simulink model "Library"  (R2020b)
settings: Solver=VariableStepAuto  StartTime=0.0  StopTime=2  RelTol=1e-3
settings Model: Creator=Stefano  LastModifiedBy=stefanopanzieri
settings SFSimCC: CustomCodeUndefinedFunction=UseInterfaceOnly

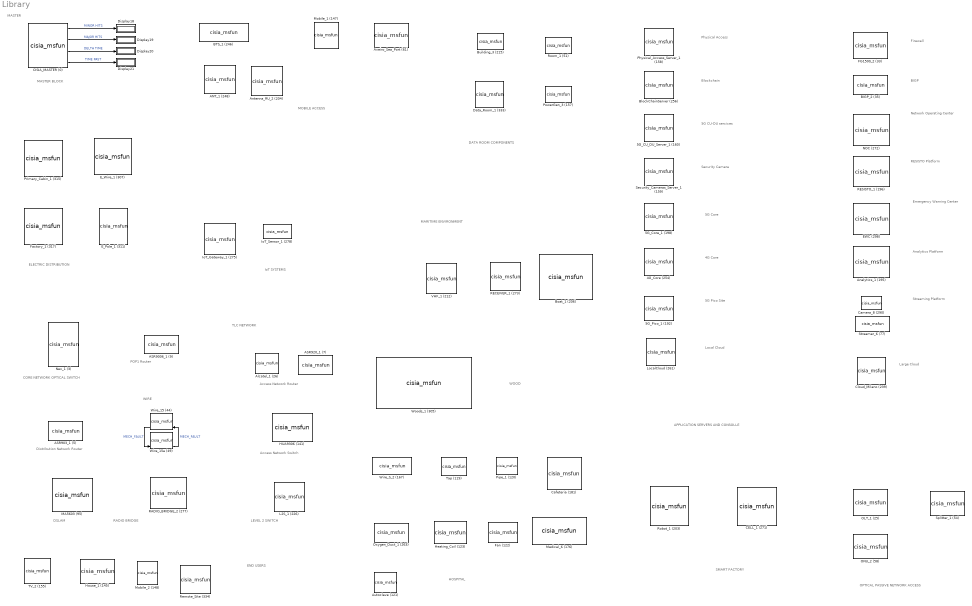
== system Library ==
  note: MASTER BLOCK
  note: MASTER
  note: ELECTRIC DISTRIBUTION
  note: TLC NETWORK
  note: MOBILE ACCESS
  note: MARITIME ENVIRONMENT
  note: DATA ROOM COMPONENTS
  note: APPLICATION SERVERS AND CONSOLLE
  note: IoT SYSTEMS
  note: SMART FACTORY
  note: HOSPITAL
  note: END USERS
  note: Access Network Router
  note: Access Network Switch
  note: Distribution Network Router
  note: DSLAM
  note: RADIO BRIDGE
  note: WIRE
  note: CORE NETWORK OPTICAL SWITCH
  note: POP1 Router
  note: LEVEL 2 SWITCH
  note: WOOD
  note: OPTICAL PASSIVE NETWORK ACCESS
  note: Physical Access
  note: Blockchain
  note: 5G CU-DU sercices
  note: Security Camera
  note: 5G Pico Site
  note: Large Cloud
  note: Local Cloud
  note: Firewall
  note: BIGP
  note: Network Operating Center
  note: RESISTO Platform
  note: Emergency Warning Center
  note: Analytics Platform
  note: Streaming Platform
  note: 4G Core
  note: 5G Core
  4G_Core (254) : M-S-Function  FunctionName=cisia_msfun  Parameters=Parameter1, Parameter2, Parameter3, resources, Parameter10, codeupdate, step_received, step_computed, dynamic_computed, step_sended, id_entity, id_project, id_type, name_type, color  mask(S-function:msfcn_unit_delay){Parameter1='4G_Core', Parameter2=1, Parameter3='ORO', resources=, Parameter10=off, codeupdate=off, step_received=|, step_computed=, dynamic_computed=, step_sended=|, id_entity=254, id_project=6, id_type=40, name_type=App_Server, color=#00AAFF}
      mask step_received=|
      | Connection=max(Connection_init,TLC_CONN);
      | TLC_services=max(TLC_services_init,TLC_SERVICE);
      | TLC_services=mod(TLC_services,10);
      | TLC_revoke=floor(TLC_SERVICE/10);
      |
      | Mechanical_Fault=max([Mechanical_Fault Mechanical_Fault_init]);
      |
      | %if strcmp(name_entity,"BlockChainServer") && (cisia.major_time>=2)
      |  % Dos_attack=1;
      |  %TLC_revoke(9)=1;
      |  %TLC_services(9)=0;
      | %end
      |
      |
      | Cyber_Fault=max(CYBER_FAULT, transpose([Dos_attack   MITM_attack Virus_Attack Port_Scan_Attack  BGP_hijacking BotNet_Attack Data_Corruption SW_Change Config_Change Port_Saturation]));
      |
      | Service_Fault=max(abs(Consumed_Services.*TLC_services-Consumed_Services));
      | Redundancy_Fault=max(abs(Consumed_Services.*TLC_CONN-Consumed_Services));
      |
      | Conn_Fault=max([Dos_attack  Mechanical_Fault  1-POWER 1-ROOM_QoS] );
      |
      |
      | Operative_Level=(1-Conn_Fault)*(1-0.5*max(Cyber_Fault))*(1-Service_Fault)*max(max(TLC_CONN),0.5);
      mask step_sended=|
      | TLC_CONN=Connection*(1-Conn_Fault);
      | TLC_SERVICE=TLC_services*(1-Conn_Fault)*(1-Service_Fault)*(1-syslog_adm_login)+10*TLC_revoke;
      | CYBER_FAULT=Cyber_Fault*(1-Conn_Fault);
      mask prompts: Parameter1 "entity name"; Parameter2 "sampling time"; Parameter3 "project"; resources "input resources and state variables"; Parameter10 "Bring state variables to output"; codeupdate "update code from mask"
      mask help: This is a level-2 MATLAB file S-function which demonstrates CISIA entity
      mask DialogControl Container1 Prompt: All parameters
      mask Display: image('Icons/App_Server.png')
  5G_CU_DU_Server_1 (160) : M-S-Function  FunctionName=cisia_msfun  Parameters=Parameter1, Parameter2, Parameter3, resources, Parameter10, codeupdate, step_received, step_computed, dynamic_computed, step_sended, id_entity, id_project, id_type, name_type, color  mask(S-function:msfcn_unit_delay){Parameter1='5G_CU_DU_Server_1', Parameter2=1, Parameter3='ORO', resources=, Parameter10=off, codeupdate=off, step_received=|, step_computed=, dynamic_computed=, step_sended=|, id_entity=160, id_project=6, id_type=40, name_type=App_Server, color=#00AAFF}
      mask step_received=|
      | Connection=max(Connection_init,TLC_CONN);
      | TLC_services=max(TLC_services_init,TLC_SERVICE);
      | TLC_services=mod(TLC_services,10);
      | TLC_revoke=floor(TLC_SERVICE/10);
      |
      | Mechanical_Fault=max([Mechanical_Fault Mechanical_Fault_init]);
      |
      | %if strcmp(name_entity,"BlockChainServer") && (cisia.major_time>=2)
      |  % Dos_attack=1;
      |  %TLC_revoke(9)=1;
      |  %TLC_services(9)=0;
      | %end
      |
      |
      | Cyber_Fault=max(CYBER_FAULT, transpose([Dos_attack   MITM_attack Virus_Attack Port_Scan_Attack  BGP_hijacking BotNet_Attack Data_Corruption SW_Change Config_Change Port_Saturation]));
      |
      | Service_Fault=max(abs(Consumed_Services.*TLC_services-Consumed_Services));
      | Redundancy_Fault=max(abs(Consumed_Services.*TLC_CONN-Consumed_Services));
      |
      | Conn_Fault=max([Dos_attack  Mechanical_Fault  1-POWER 1-ROOM_QoS] );
      |
      |
      | Operative_Level=(1-Conn_Fault)*(1-0.5*max(Cyber_Fault))*(1-Service_Fault)*max(max(TLC_CONN),0.5);
      mask step_sended=|
      | TLC_CONN=Connection*(1-Conn_Fault);
      | TLC_SERVICE=TLC_services*(1-Conn_Fault)*(1-Service_Fault)*(1-syslog_adm_login)+10*TLC_revoke;
      | CYBER_FAULT=Cyber_Fault*(1-Conn_Fault);
      mask prompts: Parameter1 "entity name"; Parameter2 "sampling time"; Parameter3 "project"; resources "input resources and state variables"; Parameter10 "Bring state variables to output"; codeupdate "update code from mask"
      mask help: This is a level-2 MATLAB file S-function which demonstrates CISIA entity
      mask DialogControl Container1 Prompt: All parameters
      mask Display: image('Icons/App_Server.png')
  5G_Core_1 (198) : M-S-Function  FunctionName=cisia_msfun  Parameters=Parameter1, Parameter2, Parameter3, resources, Parameter10, codeupdate, step_received, step_computed, dynamic_computed, step_sended, id_entity, id_project, id_type, name_type, color  mask(S-function:msfcn_unit_delay){Parameter1='5G_Core_1', Parameter2=1, Parameter3='ORO', resources=, Parameter10=off, codeupdate=off, step_received=|, step_computed=, dynamic_computed=, step_sended=|, id_entity=198, id_project=6, id_type=38, name_type=5G_Core, color=#E7A6FF}
      mask step_received=|
      | Connection=max(Connection_init,TLC_CONN);
      | TLC_services=max(TLC_services_init,TLC_SERVICE);
      | TLC_services=mod(TLC_services,10);
      | TLC_revoke=floor(TLC_SERVICE/10);
      | Mechanical_Fault=max([Mechanical_Fault Mechanical_Fault_init]);
      |
      | Cyber_Fault=max(CYBER_FAULT, transpose([Dos_attack   MITM_attack Virus_Attack Port_Scan_Attack  BGP_hijacking BotNet_Attack Data_Corruption SW_Change Config_Change Port_Saturation]));
      |
      |
      |
      | %if (cisia.major_time)>=2
      |    %Dos_attack=1;
      |    %TLC_services(5)=0;
      |   %TLC_revoke(5)=1;
      | %end
      |
      |
      | Conn_Fault=max([Dos_attack  Mechanical_Fault  1-POWER 1-ROOM_QoS] );
      |
      | Service_Fault=max(abs(Consumed_Services.*TLC_services-Consumed_Services));
      | Redundancy_Fault=max(abs(Consumed_Services.*TLC_CONN-Consumed_Services));
      |
      | Operative_Level=(1-Conn_Fault)*(1-0.5*max(Cyber_Fault))*(1-Service_Fault);
      mask step_sended=|
      | TLC_CONN=Connection*(1-Conn_Fault);
      | TLC_SERVICE=TLC_services*(1-Conn_Fault)*(1-Service_Fault)*(1 -syslog_adm_login)+10*TLC_revoke;
      | %TLC_SERVICE=TLC_services
      | CYBER_FAULT=Cyber_Fault*(1-Conn_Fault);
      mask prompts: Parameter1 "entity name"; Parameter2 "sampling time"; Parameter3 "project"; resources "input resources and state variables"; Parameter10 "Bring state variables to output"; codeupdate "update code from mask"
      mask help: This is a level-2 MATLAB file S-function which demonstrates CISIA entity
      mask DialogControl Container1 Prompt: All parameters
      mask Display: image('Icons/5G_Core.png')
  5G_Pico_1 (192) : M-S-Function  FunctionName=cisia_msfun  Parameters=Parameter1, Parameter2, Parameter3, resources, Parameter10, codeupdate, step_received, step_computed, dynamic_computed, step_sended, id_entity, id_project, id_type, name_type, color  mask(S-function:msfcn_unit_delay){Parameter1='5G_Pico_1', Parameter2=1, Parameter3='ORO', resources=, Parameter10=off, codeupdate=off, step_received=|, step_computed=, dynamic_computed=, step_sended=|, id_entity=192, id_project=6, id_type=42, name_type=5G_CU_DU, color=#FF00FF}
      mask step_received=|
      | Connection=max(Connection_init,TLC_CONN);
      | TLC_services=max(TLC_services_init,TLC_SERVICE);
      | TLC_services=mod(TLC_services,10);
      | TLC_revoke=floor(TLC_SERVICE/10);
      |
      | Cyber_Fault=max(CYBER_FAULT, transpose([Dos_attack   MITM_attack Virus_Attack Port_Scan_Attack  BGP_hijacking BotNet_Attack Data_Corruption SW_Change Config_Change Port_Saturation]));
      |
      | Conn_Fault=max([Dos_attack  Mechanical_Fault  1-POWER 1-ROOM_QoS] );
      |
      | Service_Fault=max(abs(Consumed_Services.*TLC_services-Consumed_Services));
      | Redundancy_Fault=max(abs(Consumed_Services.*TLC_CONN-Consumed_Services));
      |
      | Operative_Level=(1-Conn_Fault)*(1-0.5*max(Cyber_Fault))*(1-Service_Fault)*max(max(TLC_CONN),0.5);
      mask step_sended=|
      | TLC_CONN=Connection*(1-Conn_Fault);
      | TLC_SERVICE=TLC_services*(1-Conn_Fault)*(1-Service_Fault)+TLC_revoke*10;
      | CYBER_FAULT=Cyber_Fault*(1-Conn_Fault);
      mask prompts: Parameter1 "entity name"; Parameter2 "sampling time"; Parameter3 "project"; resources "input resources and state variables"; Parameter10 "Bring state variables to output"; codeupdate "update code from mask"
      mask help: This is a level-2 MATLAB file S-function which demonstrates CISIA entity
      mask DialogControl Container1 Prompt: All parameters
      mask Display: disp('5G_CU_DU')
  ANT_1 (248) : M-S-Function  FunctionName=cisia_msfun  Parameters=Parameter1, Parameter2, Parameter3, resources, Parameter10, codeupdate, step_received, step_computed, dynamic_computed, step_sended, id_entity, id_project, id_type, name_type, color  mask(S-function:msfcn_unit_delay){Parameter1='ANT_1', Parameter2=1, Parameter3='ORO', resources=, Parameter10=off, codeupdate=off, step_received=|, step_computed=, dynamic_computed=, step_sended=|, id_entity=248, id_project=6, id_type=55, name_type=BTS_ANTENNA, color=#FFFFFF}
      mask step_received=|
      | Connection=max(Connection_init,BTS_CONN);
      | TLC_services=max(TLC_services_init,TLC_SERVICE);
      | TLC_services=mod(TLC_services,10);
      | TLC_revoke=floor(TLC_SERVICE/10);
      |
      | Cyber_Fault=max(CYBER_FAULT, transpose([Dos_attack   MITM_attack Virus_Attack Port_Scan_Attack  BGP_hijacking BotNet_Attack Data_Corruption SW_Change Config_Change Port_Saturation]));
      |
      | Conn_Fault=max([Dos_attack  Mechanical_Fault  1-POWER] );
      |
      | Service_Fault=max(abs(Consumed_Services.*TLC_services-Consumed_Services));
      | Redundancy_Fault=max(abs(Consumed_Services.*BTS_CONN-Consumed_Services));
      |
      | Operative_Level=(1-Conn_Fault)*(1-0.5*max(Cyber_Fault))*(1-Service_Fault);
      |
      | %Operative_Level=(1-Conn_Fault)*((2*(1-Service_Fault)+(1-Redundancy_Fault))/3);
      | %Operative_Level=(1-Conn_Fault)*max(max(BTS_CONN),0.5)*((2*(1-Service_Fault)+(1-Redundancy_Fault))/3);
      |
      | % Il servizio utilizzato
      | %My_Service=max([(1-Service_Fault) (1-Redundancy_Fault)/2]);
      mask step_sended=|
      | R_CONN=Connection*(1-Conn_Fault);
      | TLC_SERVICE=TLC_services*(1-Conn_Fault)*(1-Service_Fault)+10*TLC_revoke;
      | CYBER_FAULT=Cyber_Fault*(1-Conn_Fault);
      mask prompts: Parameter1 "entity name"; Parameter2 "sampling time"; Parameter3 "project"; resources "input resources and state variables"; Parameter10 "Bring state variables to output"; codeupdate "update code from mask"
      mask help: This is a level-2 MATLAB file S-function which demonstrates CISIA entity
      mask DialogControl Container1 Prompt: All parameters
      mask Display: image('Icons/BTS_ANTENNA.png')
  ASR9006_1 (9) : M-S-Function  FunctionName=cisia_msfun  Parameters=Parameter1, Parameter2, Parameter3, resources, Parameter10, codeupdate, step_received, step_computed, dynamic_computed, step_sended, id_entity, id_project, id_type, name_type, color  mask(S-function:msfcn_unit_delay){Parameter1='ASR9006_1', Parameter2=1, Parameter3='ORO', resources=, Parameter10=off, codeupdate=off, step_received=|, step_computed=, dynamic_computed=, step_sended=|, id_entity=9, id_project=6, id_type=3, name_type=CISCO_router, color=#4DBEEE}
      mask step_received=|
      | Connection=max(Connection_init,TLC_CONN);
      | TLC_services=max(TLC_services_init,TLC_SERVICE);
      | TLC_services=mod(TLC_services,10);
      | TLC_revoke=floor(TLC_SERVICE/10);
      |
      | Cyber_Fault=max(CYBER_FAULT, transpose([Dos_attack   MITM_attack Virus_Attack Port_Scan_Attack  BGP_hijacking BotNet_Attack Data_Corruption SW_Change Config_Change Port_Saturation]));
      |
      |
      | Conn_Fault=max([Dos_attack BGP_hijacking Route_Poisoning Interface_Down Mechanical_Fault  1-POWER 1-ROOM_QoS Earthquake_Fault] );
      |
      | Room_Fault=1-ROOM_QoS;
      |
      | Operative_Level=(1-Room_Fault)*(1-Conn_Fault)*max(max(TLC_services),0.5)*(1-0.5*max(Cyber_Fault));
      mask step_sended=|
      | TLC_CONN=Connection*(1-Conn_Fault);
      | TLC_SERVICE=TLC_services*(1-Room_Fault)*(1-Conn_Fault)*(1-syslog_adm_login)+10*TLC_revoke;
      |
      |
      | Cyber_Transmitted=min(Cyber_Fault, transpose([0 0 1 0 1 1 0 0 0 1]));
      |
      | CYBER_FAULT=Cyber_Transmitted*(1-Conn_Fault);
      |
      | ROUTING_QoS=Operative_Level;
      mask prompts: Parameter1 "entity name"; Parameter2 "sampling time"; Parameter3 "project"; resources "input resources and state variables"; Parameter10 "Bring state variables to output"; codeupdate "update code from mask"
      mask help: This is a level-2 MATLAB file S-function which demonstrates CISIA entity
      mask DialogControl Container1 Prompt: All parameters
      mask Display: image('Icons/CISCO_router.png')
  ASR903_1 (5) : M-S-Function  FunctionName=cisia_msfun  Parameters=Parameter1, Parameter2, Parameter3, resources, Parameter10, codeupdate, step_received, step_computed, dynamic_computed, step_sended, id_entity, id_project, id_type, name_type, color  mask(S-function:msfcn_unit_delay){Parameter1='ASR903_1', Parameter2=1, Parameter3='ORO', resources=, Parameter10=off, codeupdate=off, step_received=|, step_computed=, dynamic_computed=, step_sended=|, id_entity=5, id_project=6, id_type=3, name_type=CISCO_router, color=#4DBEEE}
      mask step_received=|
      | Connection=max(Connection_init,TLC_CONN);
      | TLC_services=max(TLC_services_init,TLC_SERVICE);
      | TLC_services=mod(TLC_services,10);
      | TLC_revoke=floor(TLC_SERVICE/10);
      |
      | Cyber_Fault=max(CYBER_FAULT, transpose([Dos_attack   MITM_attack Virus_Attack Port_Scan_Attack  BGP_hijacking BotNet_Attack Data_Corruption SW_Change Config_Change Port_Saturation]));
      |
      |
      | Conn_Fault=max([Dos_attack BGP_hijacking Route_Poisoning Interface_Down Mechanical_Fault  1-POWER 1-ROOM_QoS Earthquake_Fault] );
      |
      | Room_Fault=1-ROOM_QoS;
      |
      | Operative_Level=(1-Room_Fault)*(1-Conn_Fault)*max(max(TLC_services),0.5)*(1-0.5*max(Cyber_Fault));
      mask step_sended=|
      | TLC_CONN=Connection*(1-Conn_Fault);
      | TLC_SERVICE=TLC_services*(1-Room_Fault)*(1-Conn_Fault)*(1-syslog_adm_login)+10*TLC_revoke;
      |
      |
      | Cyber_Transmitted=min(Cyber_Fault, transpose([0 0 1 0 1 1 0 0 0 1]));
      |
      | CYBER_FAULT=Cyber_Transmitted*(1-Conn_Fault);
      |
      | ROUTING_QoS=Operative_Level;
      mask prompts: Parameter1 "entity name"; Parameter2 "sampling time"; Parameter3 "project"; resources "input resources and state variables"; Parameter10 "Bring state variables to output"; codeupdate "update code from mask"
      mask help: This is a level-2 MATLAB file S-function which demonstrates CISIA entity
      mask DialogControl Container1 Prompt: All parameters
      mask Display: image('Icons/CISCO_router.png')
  ASR920_1 (7) : M-S-Function  FunctionName=cisia_msfun  Parameters=Parameter1, Parameter2, Parameter3, resources, Parameter10, codeupdate, step_received, step_computed, dynamic_computed, step_sended, id_entity, id_project, id_type, name_type, color  mask(S-function:msfcn_unit_delay){Parameter1='ASR920_1', Parameter2=1, Parameter3='ORO', resources=, Parameter10=off, codeupdate=off, step_received=|, step_computed=, dynamic_computed=, step_sended=|, id_entity=7, id_project=6, id_type=3, name_type=CISCO_router, color=#4DBEEE}
      mask step_received=|
      | Connection=max(Connection_init,TLC_CONN);
      | TLC_services=max(TLC_services_init,TLC_SERVICE);
      | TLC_services=mod(TLC_services,10);
      | TLC_revoke=floor(TLC_SERVICE/10);
      |
      | Cyber_Fault=max(CYBER_FAULT, transpose([Dos_attack   MITM_attack Virus_Attack Port_Scan_Attack  BGP_hijacking BotNet_Attack Data_Corruption SW_Change Config_Change Port_Saturation]));
      |
      |
      | Conn_Fault=max([Dos_attack BGP_hijacking Route_Poisoning Interface_Down Mechanical_Fault  1-POWER 1-ROOM_QoS Earthquake_Fault] );
      |
      | Room_Fault=1-ROOM_QoS;
      |
      | Operative_Level=(1-Room_Fault)*(1-Conn_Fault)*max(max(TLC_services),0.5)*(1-0.5*max(Cyber_Fault));
      mask step_sended=|
      | TLC_CONN=Connection*(1-Conn_Fault);
      | TLC_SERVICE=TLC_services*(1-Room_Fault)*(1-Conn_Fault)*(1-syslog_adm_login)+10*TLC_revoke;
      |
      |
      | Cyber_Transmitted=min(Cyber_Fault, transpose([0 0 1 0 1 1 0 0 0 1]));
      |
      | CYBER_FAULT=Cyber_Transmitted*(1-Conn_Fault);
      |
      | ROUTING_QoS=Operative_Level;
      mask prompts: Parameter1 "entity name"; Parameter2 "sampling time"; Parameter3 "project"; resources "input resources and state variables"; Parameter10 "Bring state variables to output"; codeupdate "update code from mask"
      mask help: This is a level-2 MATLAB file S-function which demonstrates CISIA entity
      mask DialogControl Container1 Prompt: All parameters
      mask Display: image('Icons/CISCO_router.png')
  Alcatel_1 (26) : M-S-Function  FunctionName=cisia_msfun  Parameters=Parameter1, Parameter2, Parameter3, resources, Parameter10, codeupdate, step_received, step_computed, dynamic_computed, step_sended, id_entity, id_project, id_type, name_type, color  mask(S-function:msfcn_unit_delay){Parameter1='Alcatel_1', Parameter2=1, Parameter3='ORO', resources=, Parameter10=off, codeupdate=off, step_received=|, step_computed=, dynamic_computed=, step_sended=|, id_entity=26, id_project=6, id_type=5, name_type=Alcatel7750, color=#ACBD7E}
      mask step_received=|
      | Connection=max(Connection_init,TLC_CONN);
      | TLC_services=max(TLC_services_init,TLC_SERVICE);
      | TLC_services=mod(TLC_services,10);
      | TLC_revoke=floor(TLC_SERVICE/10);
      |
      | Cyber_Fault=max(CYBER_FAULT, transpose([Dos_attack   MITM_attack Virus_Attack Port_Scan_Attack  BGP_hijacking BotNet_Attack Data_Corruption SW_Change Config_Change Port_Saturation]));
      |
      | Conn_Fault=max([Dos_attack  Mechanical_Fault  1-POWER 1-ROOM_QoS] );
      |
      |
      | Operative_Level=(1-Conn_Fault)*(1-0.5*max(Cyber_Fault))*max(max(TLC_services),0.5);
      mask step_sended=|
      | TLC_CONN=Connection*(1-Conn_Fault);
      | TLC_SERVICE=TLC_services*(1-Conn_Fault)+TLC_revoke*10;
      | CYBER_FAULT=Cyber_Fault*(1-Conn_Fault);
      |
      | ROUTING_QoS=Operative_Level;
      mask prompts: Parameter1 "entity name"; Parameter2 "sampling time"; Parameter3 "project"; resources "input resources and state variables"; Parameter10 "Bring state variables to output"; codeupdate "update code from mask"
      mask help: This is a level-2 MATLAB file S-function which demonstrates CISIA entity
      mask DialogControl Container1 Prompt: All parameters
      mask Display: image('Icons/Alcatel7750.png')
  Analytics_1 (195) : M-S-Function  FunctionName=cisia_msfun  Parameters=Parameter1, Parameter2, Parameter3, resources, Parameter10, codeupdate, step_received, step_computed, dynamic_computed, step_sended, id_entity, id_project, id_type, name_type, color  mask(S-function:msfcn_unit_delay){Parameter1='Analytics_1', Parameter2=1, Parameter3='ORO', resources=, Parameter10=off, codeupdate=off, step_received=|, step_computed=, dynamic_computed=, step_sended=WORKSTATION_QoS=Operative_Level;, id_entity=195, id_project=6, id_type=43, name_type=Workstation, color=#FFFFFF}
      mask step_received=|
      | Connection=max(Connection_init,TLC_CONN);
      |
      | Cyber_Fault=max(CYBER_FAULT, transpose([Dos_attack   MITM_attack Virus_Attack Port_Scan_Attack  BGP_hijacking BotNet_Attack Data_Corruption SW_Change Config_Change Port_Saturation]));
      |
      | % Vale 1 in presenza di fault
      | Conn_Fault=max([Dos_attack  Mechanical_Fault  1-POWER] );
      |
      |
      |
      | Operative_Level=(1-Conn_Fault)*max(max(TLC_CONN),0.5);
      mask prompts: Parameter1 "entity name"; Parameter2 "sampling time"; Parameter3 "project"; resources "input resources and state variables"; Parameter10 "Bring state variables to output"; codeupdate "update code from mask"
      mask help: This is a level-2 MATLAB file S-function which demonstrates CISIA entity
      mask DialogControl Container1 Prompt: All parameters
      mask Display: image('Icons/Analytics_1.png')
  Antenna_RU_2 (204) : M-S-Function  FunctionName=cisia_msfun  Parameters=Parameter1, Parameter2, Parameter3, resources, Parameter10, codeupdate, step_received, step_computed, dynamic_computed, step_sended, id_entity, id_project, id_type, name_type, color  mask(S-function:msfcn_unit_delay){Parameter1='Antenna_RU_2', Parameter2=1, Parameter3='ORO', resources=, Parameter10=off, codeupdate=off, step_received=|, step_computed=, dynamic_computed=, step_sended=|, id_entity=204, id_project=6, id_type=41, name_type=RU_ANTENNA, color=#FFFFFF}
      mask step_received=|
      | Connection=max(Connection_init,TLC_CONN);
      | TLC_services=max(TLC_services_init,TLC_SERVICE);
      | TLC_services=mod(TLC_services,10);
      | TLC_revoke=floor(TLC_SERVICE/10);
      |
      | Cyber_Fault=max(CYBER_FAULT, transpose([Dos_attack   MITM_attack Virus_Attack Port_Scan_Attack  BGP_hijacking BotNet_Attack Data_Corruption SW_Change Config_Change Port_Saturation]));
      |
      | % Vale 1 in presenza di fault
      | Conn_Fault=max([Dos_attack  Mechanical_Fault  1-POWER] );
      |
      | Service_Fault=max(abs(Consumed_Services.*TLC_services-Consumed_Services));
      | Redundancy_Fault=max(abs(Consumed_Services.*TLC_CONN-Consumed_Services));
      |
      |
      | Operative_Level=(1-Conn_Fault)*max(max(TLC_services),0.5)*(1-Service_Fault)*(1-0.5*max(Cyber_Fault))*max(max(TLC_CONN),0.5);
      |
      | % Il servizio utilizzato
      | %My_Service=max([(1-Service_Fault) (1-Redundancy_Fault)/2]);
      mask step_sended=|
      | R_CONN=Connection*(1-Conn_Fault);
      | TLC_SERVICE=TLC_services*(1-Conn_Fault)+10*TLC_revoke;
      |
      | Cyber_Transmitted=min(Cyber_Fault, transpose([0 0 1 0 1 1 0 0 0 1]));
      | CYBER_FAULT=Cyber_Transmitted*(1-Conn_Fault);
      mask prompts: Parameter1 "entity name"; Parameter2 "sampling time"; Parameter3 "project"; resources "input resources and state variables"; Parameter10 "Bring state variables to output"; codeupdate "update code from mask"
      mask help: This is a level-2 MATLAB file S-function which demonstrates CISIA entity
      mask DialogControl Container1 Prompt: All parameters
      mask Display: image('Icons/RU_ANTENNA.png')
  Autoclave (121) : M-S-Function  FunctionName=cisia_msfun  Parameters=Parameter1, Parameter2, Parameter3, resources, Parameter10, codeupdate, step_received, step_computed, dynamic_computed, step_sended, id_entity, id_project, id_type, name_type, color  mask(S-function:msfcn_unit_delay){Parameter1='Autoclave', Parameter2=1, Parameter3='ORO', resources=, Parameter10=off, codeupdate=off, step_received=|, step_computed=, dynamic_computed=, step_sended=WATER=Operative_Level;, id_entity=121, id_project=6, id_type=33, name_type=Autoclave, color=#FFFFFF}
      mask step_received=|
      | Water_Fault=1-WATER;
      | Power_Fault=1-POWER;
      |
      | Operative_Level=min([ 1-Mechanical_Fault 1-Power_Fault 1-Water_Fault]);
      mask prompts: Parameter1 "entity name"; Parameter2 "sampling time"; Parameter3 "project"; resources "input resources and state variables"; Parameter10 "Bring state variables to output"; codeupdate "update code from mask"
      mask help: This is a level-2 MATLAB file S-function which demonstrates CISIA entity
      mask DialogControl Container1 Prompt: All parameters
      mask Display: disp('Autoclave')
  Aveiro_Sea_Port (61) : M-S-Function  FunctionName=cisia_msfun  Parameters=Parameter1, Parameter2, Parameter3, resources, Parameter10, codeupdate, step_received, step_computed, dynamic_computed, step_sended, id_entity, id_project, id_type, name_type, color  mask(S-function:msfcn_unit_delay){Parameter1='Aveiro_Sea_Port', Parameter2=1, Parameter3='ORO', resources=, Parameter10=off, codeupdate=off, step_received=|, step_computed=, dynamic_computed=, step_sended=|, id_entity=61, id_project=6, id_type=14, name_type=Cell_Area, color=#0FFFFF}
      mask step_received=|
      | Connection=max(Connection_init,R_CONN);
      | TLC_services=max(TLC_services_init,TLC_SERVICE);
      | TLC_services=mod(TLC_services,10);
      | TLC_revoke=floor(TLC_SERVICE/10);
      |
      | Cyber_Fault=max(CYBER_FAULT, transpose([Dos_attack   MITM_attack Virus_Attack Port_Scan_Attack  BGP_hijacking BotNet_Attack Data_Corruption SW_Change Config_Change Port_Saturation]));
      |
      | % Vale 1 in presenza di fault
      | Conn_Fault=max([Dos_attack  Mechanical_Fault] );
      |
      | Service_Fault=max(abs(Consumed_Services.*TLC_services-Consumed_Services));
      | Redundancy_Fault=max(abs(Consumed_Services.*R_CONN-Consumed_Services));
      |
      |
      | Operative_Level=(1-Conn_Fault)*max(max(R_CONN),0.5)*((2*(1-Service_Fault)+(1-Redundancy_Fault))/3);
      |
      | % Il servizio utilizzato
      | My_Service=max([(1-Service_Fault) (1-Redundancy_Fault)/2]);
      mask step_sended=|
      | R_CONN=Connection*(1-Conn_Fault);
      | TLC_SERVICE=TLC_services*(1-Conn_Fault)+10*TLC_revoke;
      | CYBER_FAULT=Cyber_Fault*(1-Conn_Fault);
      |
      | CELL_QoS=My_Service;
      mask prompts: Parameter1 "entity name"; Parameter2 "sampling time"; Parameter3 "project"; resources "input resources and state variables"; Parameter10 "Bring state variables to output"; codeupdate "update code from mask"
      mask help: This is a level-2 MATLAB file S-function which demonstrates CISIA entity
      mask DialogControl Container1 Prompt: All parameters
      mask Display: disp('Cell_Area')
  BIGP_2 (35) : M-S-Function  FunctionName=cisia_msfun  Parameters=Parameter1, Parameter2, Parameter3, resources, Parameter10, codeupdate, step_received, step_computed, dynamic_computed, step_sended, id_entity, id_project, id_type, name_type, color  mask(S-function:msfcn_unit_delay){Parameter1='BIGP_2', Parameter2=1, Parameter3='ORO', resources=, Parameter10=off, codeupdate=off, step_received=|, step_computed=, dynamic_computed=, step_sended=|, id_entity=35, id_project=6, id_type=7, name_type=F5BIGP, color=#0072BD}
      mask step_received=|
      | Connection=max(Connection_init,TLC_CONN);
      | TLC_services=max(TLC_services_init,TLC_SERVICE);
      | TLC_services=mod(TLC_services,10);
      | TLC_revoke=floor(TLC_SERVICE/10);
      |
      | Cyber_Fault=max(CYBER_FAULT, transpose([Dos_attack   MITM_attack Virus_Attack Port_Scan_Attack  BGP_hijacking BotNet_Attack Data_Corruption SW_Change Config_Change Port_Saturation]));
      |
      | Conn_Fault=max([Dos_attack  Mechanical_Fault  1-POWER 1-ROOM_QoS] );
      |
      | Service_Fault=max(abs(Consumed_Services.*TLC_services-Consumed_Services));
      | Redundancy_Fault=max(abs(Consumed_Services.*TLC_CONN-Consumed_Services));
      |
      | %Operative_Level=(1-Conn_Fault)*((2*(1-Service_Fault)+(1-Redundancy_Fault))/3);
      | Operative_Level=(1-Conn_Fault)*(1-0.5*max(Cyber_Fault))*(1-Service_Fault)*max(max(TLC_CONN),0.5);
      mask step_sended=|
      | TLC_CONN=Connection*(1-Conn_Fault);
      | TLC_SERVICE=TLC_services*(1-Conn_Fault)*(1-Service_Fault)+10*TLC_revoke;
      |
      | Cyber_Transmitted=min(Cyber_Fault, transpose([0 0 1 0 1 1 0 0 0 1]));
      |
      | CYBER_FAULT=Cyber_Transmitted*(1-Conn_Fault);
      mask prompts: Parameter1 "entity name"; Parameter2 "sampling time"; Parameter3 "project"; resources "input resources and state variables"; Parameter10 "Bring state variables to output"; codeupdate "update code from mask"
      mask help: This is a level-2 MATLAB file S-function which demonstrates CISIA entity
      mask DialogControl Container1 Prompt: All parameters
      mask Display: disp('F5BIGP')
  BTS_1 (246) : M-S-Function  FunctionName=cisia_msfun  Parameters=Parameter1, Parameter2, Parameter3, resources, Parameter10, codeupdate, step_received, step_computed, dynamic_computed, step_sended, id_entity, id_project, id_type, name_type, color  mask(S-function:msfcn_unit_delay){Parameter1='BTS_1', Parameter2=1, Parameter3='ORO', resources=, Parameter10=off, codeupdate=off, step_received=|, step_computed=, dynamic_computed=, step_sended=|, id_entity=246, id_project=6, id_type=54, name_type=BaseTransceiverStation, color=#FFFFFF}
      mask step_received=|
      | Connection=max(Connection_init,TLC_CONN);
      | TLC_services=max(TLC_services_init,TLC_SERVICE);
      | TLC_services=mod(TLC_services,10);
      | TLC_revoke=floor(TLC_SERVICE/10);
      |
      | Cyber_Fault=max(CYBER_FAULT, transpose([Dos_attack   MITM_attack Virus_Attack Port_Scan_Attack  BGP_hijacking BotNet_Attack Data_Corruption SW_Change Config_Change Port_Saturation]));
      |
      | Conn_Fault=max([Dos_attack  Mechanical_Fault ] );
      |
      | Operative_Level=(1-Conn_Fault)*max(max(TLC_services),0.5)*(1-0.5*max(Cyber_Fault));
      mask step_sended=|
      | BTS_CONN=Connection*(1-Conn_Fault);
      | TLC_SERVICE=TLC_services*(1-Conn_Fault)+10*TLC_revoke;
      | CYBER_FAULT=Cyber_Fault*(1-Conn_Fault);
      mask prompts: Parameter1 "entity name"; Parameter2 "sampling time"; Parameter3 "project"; resources "input resources and state variables"; Parameter10 "Bring state variables to output"; codeupdate "update code from mask"
      mask help: This is a level-2 MATLAB file S-function which demonstrates CISIA entity
      mask DialogControl Container1 Prompt: All parameters
      mask Display: disp('BaseTransceiverStation')
  BlockChainServer (256) : M-S-Function  FunctionName=cisia_msfun  Parameters=Parameter1, Parameter2, Parameter3, resources, Parameter10, codeupdate, step_received, step_computed, dynamic_computed, step_sended, id_entity, id_project, id_type, name_type, color  mask(S-function:msfcn_unit_delay){Parameter1='BlockChainServer', Parameter2=1, Parameter3='ORO', resources=, Parameter10=on, codeupdate=off, step_received=|, step_computed=, dynamic_computed=, step_sended=|, id_entity=256, id_project=6, id_type=40, name_type=App_Server, color=#00AAFF}
      mask step_received=|
      | Connection=max(Connection_init,TLC_CONN);
      | TLC_services=max(TLC_services_init,TLC_SERVICE);
      | TLC_services=mod(TLC_services,10);
      | TLC_revoke=floor(TLC_SERVICE/10);
      |
      | Mechanical_Fault=max([Mechanical_Fault Mechanical_Fault_init]);
      |
      | %if strcmp(name_entity,"BlockChainServer") && (cisia.major_time>=2)
      |  % Dos_attack=1;
      |  %TLC_revoke(9)=1;
      |  %TLC_services(9)=0;
      | %end
      |
      |
      | Cyber_Fault=max(CYBER_FAULT, transpose([Dos_attack   MITM_attack Virus_Attack Port_Scan_Attack  BGP_hijacking BotNet_Attack Data_Corruption SW_Change Config_Change Port_Saturation]));
      |
      | Service_Fault=max(abs(Consumed_Services.*TLC_services-Consumed_Services));
      | Redundancy_Fault=max(abs(Consumed_Services.*TLC_CONN-Consumed_Services));
      |
      | Conn_Fault=max([Dos_attack  Mechanical_Fault  1-POWER 1-ROOM_QoS] );
      |
      |
      | Operative_Level=(1-Conn_Fault)*(1-0.5*max(Cyber_Fault))*(1-Service_Fault)*max(max(TLC_CONN),0.5);
      mask step_sended=|
      | TLC_CONN=Connection*(1-Conn_Fault);
      | TLC_SERVICE=TLC_services*(1-Conn_Fault)*(1-Service_Fault)*(1-syslog_adm_login)+10*TLC_revoke;
      | CYBER_FAULT=Cyber_Fault*(1-Conn_Fault);
      mask prompts: Parameter1 "entity name"; Parameter2 "sampling time"; Parameter3 "project"; resources "input resources and state variables"; Parameter10 "Bring state variables to output"; codeupdate "update code from mask"
      mask help: This is a level-2 MATLAB file S-function which demonstrates CISIA entity
      mask DialogControl Container1 Prompt: All parameters
      mask Display: image('Icons/App_Server.png')
  Boat_1 (206) : M-S-Function  FunctionName=cisia_msfun  Parameters=Parameter1, Parameter2, Parameter3, resources, Parameter10, codeupdate, step_received, step_computed, dynamic_computed, step_sended, id_entity, id_project, id_type, name_type, color  mask(S-function:msfcn_unit_delay){Parameter1='Boat_1', Parameter2=1, Parameter3='ORO', resources=, Parameter10=off, codeupdate=off, step_received=|, step_computed=, dynamic_computed=, step_sended=|, id_entity=206, id_project=6, id_type=45, name_type=Boat, color=#FFFFFF}
      mask step_received=|
      | Conn_Fault=1-max(VDES_CONN,AIS_CONN);
      |
      |
      | Operative_Level=(1-Mechanical_Fault)*(1-Conn_Fault);
      mask step_sended=|
      | BOAT_QoS=Operative_Level;
      | AIS_CON=1-Conn_Fault;
      | VDES_CONN=1-Conn_Fault;
      mask prompts: Parameter1 "entity name"; Parameter2 "sampling time"; Parameter3 "project"; resources "input resources and state variables"; Parameter10 "Bring state variables to output"; codeupdate "update code from mask"
      mask help: This is a level-2 MATLAB file S-function which demonstrates CISIA entity
      mask DialogControl Container1 Prompt: All parameters
      mask Display: image('Icons/Boat.png')
  Building_3 (215) : M-S-Function  FunctionName=cisia_msfun  Parameters=Parameter1, Parameter2, Parameter3, resources, Parameter10, codeupdate, step_received, step_computed, dynamic_computed, step_sended, id_entity, id_project, id_type, name_type, color  mask(S-function:msfcn_unit_delay){Parameter1='Building_3', Parameter2=1, Parameter3='ORO', resources=, Parameter10=off, codeupdate=off, step_received=|, step_computed=, dynamic_computed=, step_sended=|, id_entity=215, id_project=6, id_type=10, name_type=Building, color=#AB7A07}
      mask step_received=|
      | Physical_Fault=max([Unauthorized_Access Perimeter_Security_Fault Security_Camera_Fault Earthquake_Fault]);
      |
      | Conn_Fault=max([Power_Fault 1-ROOM_QoS]);
      |
      | Operative_Level=min([ (1-Physical_Fault) (1-Conn_Fault) (1-Perimeter_Security_Fault) (1-Earthquake_Fault) ]);
      mask step_sended=|
      | BUILDING_QoS=Operative_Level;
      |
      | %Cyber_Fault=0.3*ones(size(Cyber_Fault));
      |
      | CYBER_FAULT=Perimeter_Security_Fault*Cyber_Fault;
      mask prompts: Parameter1 "entity name"; Parameter2 "sampling time"; Parameter3 "project"; resources "input resources and state variables"; Parameter10 "Bring state variables to output"; codeupdate "update code from mask"
      mask help: This is a level-2 MATLAB file S-function which demonstrates CISIA entity
      mask DialogControl Container1 Prompt: All parameters
      mask Display: image('Icons/Building.png')
  CELL_1 (271) : M-S-Function  FunctionName=cisia_msfun  Parameters=Parameter1, Parameter2, Parameter3, resources, Parameter10, codeupdate, step_received, step_computed, dynamic_computed, step_sended, id_entity, id_project, id_type, name_type, color  mask(S-function:msfcn_unit_delay){Parameter1='CELL_1', Parameter2=1, Parameter3='ORO', resources=, Parameter10=off, codeupdate=off, step_received=Operative_Level=ROBOT_QoS;, step_computed=, dynamic_computed=, step_sended=WORKING_CELL_QoS=Operative_Level;, id_entity=271, id_project=6, id_type=58, name_type=Working_Cell, color=#00FFAA}
      mask prompts: Parameter1 "entity name"; Parameter2 "sampling time"; Parameter3 "project"; resources "input resources and state variables"; Parameter10 "Bring state variables to output"; codeupdate "update code from mask"
      mask help: This is a level-2 MATLAB file S-function which demonstrates CISIA entity
      mask DialogControl Container1 Prompt: All parameters
      mask Display: image('Icons/Working_Cell.png')
  CISIA_MASTER (0) : M-S-Function  FunctionName=cisia_msfun  Parameters=Parameter1, Parameter2, Parameter3, resources, Parameter4, Parameter5, Parameter6, Parameter7, Parameter8, Parameter9  mask(S-function:msfcn_unit_delay){Parameter1='CISIA_MASTER', Parameter2=0.001, Parameter3='ORO', resources=off, Parameter4=on, Parameter5=off, Parameter6=off, Parameter7=off, Parameter8=1, Parameter9=off}
      mask prompts: Parameter1 "entity name"; Parameter2 "sampling time"; Parameter3 "project"; resources "Save status at each major hit"; Parameter4 "Show Operative Levels with colors"; Parameter5 "Load Entities from file"; Parameter6 "Load Start from Mask"; Parameter7 "Real Time"; Parameter8 "Real Time Hit (sec)"; Parameter9 "Skip saving"
      mask help: This is a level-2 MATLAB file S-function which demonstrates CISIA entity
      mask Display: disp('MASTER BLOCK')
  Cafeteria (181) : M-S-Function  FunctionName=cisia_msfun  Parameters=Parameter1, Parameter2, Parameter3, resources, Parameter10, codeupdate, step_received, step_computed, dynamic_computed, step_sended, id_entity, id_project, id_type, name_type, color  mask(S-function:msfcn_unit_delay){Parameter1='Cafeteria', Parameter2=1, Parameter3='ORO', resources=, Parameter10=off, codeupdate=off, step_received=|, step_computed=, dynamic_computed=, step_sended=ORDINARY_ROOM_QoS= Operative_Level;, id_entity=181, id_project=6, id_type=26, name_type=Ordinary_Room, color=#FFFFFF}
      mask step_received=|
      | Power_Fault=1-POWER;
      | Air_Fault=1-AIR;
      |
      |
      | Operative_Level=(1-Fire_Fault)*(1-0.5*Power_Fault)*(1-0-5*Air_Fault);
      mask prompts: Parameter1 "entity name"; Parameter2 "sampling time"; Parameter3 "project"; resources "input resources and state variables"; Parameter10 "Bring state variables to output"; codeupdate "update code from mask"
      mask help: This is a level-2 MATLAB file S-function which demonstrates CISIA entity
      mask DialogControl Container1 Prompt: All parameters
      mask Display: disp('Ordinary_Room')
  Camera_8 (290) : M-S-Function  FunctionName=cisia_msfun  Parameters=Parameter1, Parameter2, Parameter3, resources, Parameter10, codeupdate, step_received, step_computed, dynamic_computed, step_sended, id_entity, id_project, id_type, name_type, color  mask(S-function:msfcn_unit_delay){Parameter1='Camera_8', Parameter2=1, Parameter3='ORO', resources=, Parameter10=off, codeupdate=off, step_received=, step_computed=, dynamic_computed=, step_sended=STREAM=Stream_source;, id_entity=290, id_project=6, id_type=52, name_type=Camera, color=#FFFFFF}
      mask prompts: Parameter1 "entity name"; Parameter2 "sampling time"; Parameter3 "project"; resources "input resources and state variables"; Parameter10 "Bring state variables to output"; codeupdate "update code from mask"
      mask help: This is a level-2 MATLAB file S-function which demonstrates CISIA entity
      mask DialogControl Container1 Prompt: All parameters
      mask Display: image('Icons/Camera.png')
  Cloud_Milano (239) : M-S-Function  FunctionName=cisia_msfun  Parameters=Parameter1, Parameter2, Parameter3, resources, Parameter10, codeupdate, step_received, step_computed, dynamic_computed, step_sended, id_entity, id_project, id_type, name_type, color  mask(S-function:msfcn_unit_delay){Parameter1='Cloud_Milano', Parameter2=1, Parameter3='ORO', resources=, Parameter10=off, codeupdate=off, step_received=|, step_computed=, dynamic_computed=, step_sended=|, id_entity=239, id_project=6, id_type=53, name_type=CloudServer, color=#FFFFFF}
      mask step_received=|
      | Connection=max(Connection_init,TLC_CONN);
      | TLC_services=max(TLC_services_init,TLC_SERVICE);
      | TLC_services=mod(TLC_services,10);
      | TLC_revoke=floor(TLC_SERVICE/10);
      |
      | %TLC_services=max(TLC_services_init*(1+cisia.major_time),TLC_SERVICE);
      |
      |
      | Mechanical_Fault=max([Mechanical_Fault Mechanical_Fault_init]);
      |
      | Cyber_Fault=max(CYBER_FAULT, transpose([Dos_attack   MITM_attack Virus_Attack Port_Scan_Attack  BGP_hijacking BotNet_Attack Data_Corruption SW_Change Config_Change Port_Saturation]));
      |
      | Conn_Fault=max([Dos_attack  Mechanical_Fault  1-POWER 1-ROOM_QoS] );
      |
      | Service_Fault=max(abs(Consumed_Services.*TLC_services-Consumed_Services));
      | Redundancy_Fault=max(abs(Consumed_Services.*TLC_CONN-Consumed_Services));
      |
      | Operative_Level=(1-Conn_Fault)*(1-0.5*max(Cyber_Fault))*(1-Service_Fault)*max(max(TLC_CONN),0.5);
      mask step_sended=|
      | TLC_CONN=Connection*(1-Conn_Fault);
      | TLC_SERVICE=TLC_services*(1-Conn_Fault)*(1-Service_Fault)+10*TLC_revoke;
      | CYBER_FAULT=Cyber_Fault*(1-Conn_Fault);
      mask prompts: Parameter1 "entity name"; Parameter2 "sampling time"; Parameter3 "project"; resources "input resources and state variables"; Parameter10 "Bring state variables to output"; codeupdate "update code from mask"
      mask help: This is a level-2 MATLAB file S-function which demonstrates CISIA entity
      mask DialogControl Container1 Prompt: All parameters
      mask Display: image('Icons/CloudServer.png')
  Data_Room_1 (333) : M-S-Function  FunctionName=cisia_msfun  Parameters=Parameter1, Parameter2, Parameter3, resources, Parameter10, codeupdate, step_received, step_computed, dynamic_computed, step_sended, id_entity, id_project, id_type, name_type, color  mask(S-function:msfcn_unit_delay){Parameter1='Data_Room_1', Parameter2=1, Parameter3='ORO', resources=, Parameter10=off, codeupdate=off, step_received=|, step_computed=, dynamic_computed=, step_sended=ROOM_QoS=Operative_Level;, id_entity=333, id_project=6, id_type=78, name_type=DATA_ROOM, color=#FFFFFF}
      mask step_received=|
      | Physical_Fault=max([Power_Fault Flooding_Fault Fire_Fault Cooling_Fault 1-POWER]);
      |
      |
      | Operative_Level=min([1-Power_Fault 1-Flooding_Fault  1-Fire_Fault  1-Cooling_Fault  POWER  1-USB_Device_Insertion/2 1-Unknown_Device*3/4 1-Rouge_Access 1-Config_Change 1-Unauthorized_Access/4 1-Port_Scan_Attack/2]);
      mask prompts: Parameter1 "entity name"; Parameter2 "sampling time"; Parameter3 "project"; resources "input resources and state variables"; Parameter10 "Bring state variables to output"; codeupdate "update code from mask"
      mask help: This is a level-2 MATLAB file S-function which demonstrates CISIA entity
      mask DialogControl Container1 Prompt: All parameters
      mask Display: image('Icons/DATA_ROOM.png')
  Display{18..21} (4 alike) : Display
  EWC (298) : M-S-Function  FunctionName=cisia_msfun  Parameters=Parameter1, Parameter2, Parameter3, resources, Parameter10, codeupdate, step_received, step_computed, dynamic_computed, step_sended, id_entity, id_project, id_type, name_type, color  mask(S-function:msfcn_unit_delay){Parameter1='EWC', Parameter2=1, Parameter3='ORO', resources=, Parameter10=off, codeupdate=off, step_received=|, step_computed=, dynamic_computed=, step_sended=WORKSTATION_QoS=Operative_Level;, id_entity=298, id_project=6, id_type=43, name_type=Workstation, color=#FFFFFF}
      mask step_received=|
      | Connection=max(Connection_init,TLC_CONN);
      |
      | Cyber_Fault=max(CYBER_FAULT, transpose([Dos_attack   MITM_attack Virus_Attack Port_Scan_Attack  BGP_hijacking BotNet_Attack Data_Corruption SW_Change Config_Change Port_Saturation]));
      |
      | % Vale 1 in presenza di fault
      | Conn_Fault=max([Dos_attack  Mechanical_Fault  1-POWER] );
      |
      |
      |
      | Operative_Level=(1-Conn_Fault)*max(max(TLC_CONN),0.5);
      mask prompts: Parameter1 "entity name"; Parameter2 "sampling time"; Parameter3 "project"; resources "input resources and state variables"; Parameter10 "Bring state variables to output"; codeupdate "update code from mask"
      mask help: This is a level-2 MATLAB file S-function which demonstrates CISIA entity
      mask DialogControl Container1 Prompt: All parameters
      mask Display: image('Icons/Workstation.png')
  E_Pole_1 (311) : M-S-Function  FunctionName=cisia_msfun  Parameters=Parameter1, Parameter2, Parameter3, resources, Parameter10, codeupdate, step_received, step_computed, dynamic_computed, step_sended, id_entity, id_project, id_type, name_type, color  mask(S-function:msfcn_unit_delay){Parameter1='E_Pole_1', Parameter2=1, Parameter3='ORO', resources=, Parameter10=off, codeupdate=off, step_received=|, step_computed=, dynamic_computed=, step_sended=|, id_entity=311, id_project=6, id_type=68, name_type=Electric_Pole, color=#FFFFFF}
      mask step_received=|
      | Power_Gen=max(E_POWER_1,E_POWER_2);
      |
      | Fire_Fault=FLAME;
      |
      | Physical_Fault=max(Fire_Fault,Mechanical_Fault);
      |
      | Operative_Level=1-Physical_Fault;
      mask step_sended=|
      | E_POWER_1=Power_Gen*(1-Physical_Fault);
      | E_POWER_2=Power_Gen*(1-Physical_Fault);
      mask prompts: Parameter1 "entity name"; Parameter2 "sampling time"; Parameter3 "project"; resources "input resources and state variables"; Parameter10 "Bring state variables to output"; codeupdate "update code from mask"
      mask help: This is a level-2 MATLAB file S-function which demonstrates CISIA entity
      mask DialogControl Container1 Prompt: All parameters
      mask Display: image('Icons/Electric_Pole.png')
  E_Wire_1 (307) : M-S-Function  FunctionName=cisia_msfun  Parameters=Parameter1, Parameter2, Parameter3, resources, Parameter10, codeupdate, step_received, step_computed, dynamic_computed, step_sended, id_entity, id_project, id_type, name_type, color  mask(S-function:msfcn_unit_delay){Parameter1='E_Wire_1', Parameter2=1, Parameter3='ORO', resources=, Parameter10=off, codeupdate=off, step_received=|, step_computed=, dynamic_computed=, step_sended=|, id_entity=307, id_project=6, id_type=67, name_type=Electric_Wire, color=#FFFFFF}
      mask step_received=|
      | Power_Gen=max(E_POWER_1,E_POWER_2);
      |
      | Fire_Fault=FLAME;
      |
      | Physical_Fault=max(Fire_Fault,Mechanical_Fault);
      |
      | Operative_Level=1-Physical_Fault;
      mask step_sended=|
      | E_POWER_1=Power_Gen*(1-Physical_Fault);
      | E_POWER_2=Power_Gen*(1-Physical_Fault);
      mask prompts: Parameter1 "entity name"; Parameter2 "sampling time"; Parameter3 "project"; resources "input resources and state variables"; Parameter10 "Bring state variables to output"; codeupdate "update code from mask"
      mask help: This is a level-2 MATLAB file S-function which demonstrates CISIA entity
      mask DialogControl Container1 Prompt: All parameters
      mask Display: image('Icons/Electric_Wire.png')
  FG1500_2 (33) : M-S-Function  FunctionName=cisia_msfun  Parameters=Parameter1, Parameter2, Parameter3, resources, Parameter10, codeupdate, step_received, step_computed, dynamic_computed, step_sended, id_entity, id_project, id_type, name_type, color  mask(S-function:msfcn_unit_delay){Parameter1='FG1500_2', Parameter2=1, Parameter3='ORO', resources=, Parameter10=off, codeupdate=off, step_received=|, step_computed=, dynamic_computed=, step_sended=|, id_entity=33, id_project=6, id_type=6, name_type=FortiGate1500D, color=#EDB120}
      mask step_received=|
      | Connection=max(Connection_init,TLC_CONN);
      | TLC_services=max(TLC_services_init,TLC_SERVICE);
      | TLC_services=mod(TLC_services,10);
      | TLC_revoke=floor(TLC_SERVICE/10);
      |
      | Cyber_Fault=max(CYBER_FAULT, transpose([Dos_attack   MITM_attack Virus_Attack Port_Scan_Attack  BGP_hijacking BotNet_Attack Data_Corruption SW_Change Config_Change Port_Saturation]));
      |
      | Conn_Fault=max([Dos_attack  Mechanical_Fault  1-POWER 1-ROOM_QoS  0.5*max(Cyber_Fault)] );
      |
      | Service_Fault=max(abs(Consumed_Services.*TLC_services-Consumed_Services));
      | Redundancy_Fault=max(abs(Consumed_Services.*TLC_CONN-Consumed_Services));
      |
      | %Operative_Level=(1-Conn_Fault)*((2*(1-Service_Fault)+(1-Redundancy_Fault))/3);
      | Operative_Level=(1-Conn_Fault)*(1-0.5*max(Cyber_Fault))*(1-Service_Fault)*max(max(TLC_CONN),0.5);
      mask step_sended=|
      | TLC_CONN=Connection*(1-Conn_Fault);
      | TLC_SERVICE=TLC_services*(1-Conn_Fault)*(1-Service_Fault)+10*TLC_revoke;
      |
      | Cyber_Transmitted=min(Cyber_Fault, transpose([0 0 1 0 1 1 0 0 0 1]));
      | CYBER_FAULT=Cyber_Transmitted*(1-Conn_Fault);
      |
      | FIREWALL_QoS=(1-Service_Fault)*(1-Conn_Fault);
      | REDUNDANCY_QoS=(1-Redundancy_Fault);
      mask prompts: Parameter1 "entity name"; Parameter2 "sampling time"; Parameter3 "project"; resources "input resources and state variables"; Parameter10 "Bring state variables to output"; codeupdate "update code from mask"
      mask help: This is a level-2 MATLAB file S-function which demonstrates CISIA entity
      mask DialogControl Container1 Prompt: All parameters
      mask Display: image('Icons/FortiGate1500D.png')
  Factory_1 (317) : M-S-Function  FunctionName=cisia_msfun  Parameters=Parameter1, Parameter2, Parameter3, resources, Parameter10, codeupdate, step_received, step_computed, dynamic_computed, step_sended, id_entity, id_project, id_type, name_type, color  mask(S-function:msfcn_unit_delay){Parameter1='Factory_1', Parameter2=1, Parameter3='ORO', resources=, Parameter10=off, codeupdate=off, step_received=|, step_computed=, dynamic_computed=, step_sended=E_LOAD_QoS=Operative_Level;, id_entity=317, id_project=6, id_type=69, name_type=Electric_Load, color=#FFFFFF}
      mask step_received=|
      | Power_Gen=max(Power_Gen_init,E_POWER_1);
      |
      | Physical_Fault=max([Fire_Fault  Mechanical_Fault] );
      |
      | Power_Fault=max(abs(Consumed_Power.*E_POWER_1-Consumed_Power));
      |
      |
      | Operative_Level=max([1-Power_Fault 0.5])*(1-Physical_Fault);
      mask prompts: Parameter1 "entity name"; Parameter2 "sampling time"; Parameter3 "project"; resources "input resources and state variables"; Parameter10 "Bring state variables to output"; codeupdate "update code from mask"
      mask help: This is a level-2 MATLAB file S-function which demonstrates CISIA entity
      mask DialogControl Container1 Prompt: All parameters
      mask Display: image('Icons/Factory_1.png')
  Fan (122) : M-S-Function  FunctionName=cisia_msfun  Parameters=Parameter1, Parameter2, Parameter3, resources, Parameter10, codeupdate, step_received, step_computed, dynamic_computed, step_sended, id_entity, id_project, id_type, name_type, color  mask(S-function:msfcn_unit_delay){Parameter1='Fan', Parameter2=1, Parameter3='ORO', resources=, Parameter10=off, codeupdate=off, step_received=|, step_computed=, dynamic_computed=, step_sended=AIR=Operative_Level;, id_entity=122, id_project=6, id_type=34, name_type=Fan, color=#79DE31}
      mask step_received=|
      | Power_Fault=1-POWER;
      |
      | Operative_Level=(1-Mechanical_Fault)*(1-0.5*Power_Fault);
      mask prompts: Parameter1 "entity name"; Parameter2 "sampling time"; Parameter3 "project"; resources "input resources and state variables"; Parameter10 "Bring state variables to output"; codeupdate "update code from mask"
      mask help: This is a level-2 MATLAB file S-function which demonstrates CISIA entity
      mask DialogControl Container1 Prompt: All parameters
      mask Display: disp('Fan')
  HUA9306 (141) : M-S-Function  FunctionName=cisia_msfun  Parameters=Parameter1, Parameter2, Parameter3, resources, Parameter10, codeupdate, step_received, step_computed, dynamic_computed, step_sended, id_entity, id_project, id_type, name_type, color  mask(S-function:msfcn_unit_delay){Parameter1='HUA9306', Parameter2=1, Parameter3='ORO', resources=, Parameter10=off, codeupdate=off, step_received=|, step_computed=, dynamic_computed=, step_sended=|, id_entity=141, id_project=6, id_type=22, name_type=HuaweiSwitch, color=#139FFF}
      mask step_received=|
      | Connection=max(Connection_init,TLC_CONN);
      | TLC_services=max(TLC_services_init,TLC_SERVICE);
      | TLC_services=mod(TLC_services,10);
      | TLC_revoke=floor(TLC_SERVICE/10);
      |
      | Cyber_Fault=max(CYBER_FAULT, transpose([Dos_attack   MITM_attack Virus_Attack Port_Scan_Attack  BGP_hijacking BotNet_Attack Data_Corruption SW_Change Config_Change Port_Saturation]));
      |
      | Port_Isolation=min(max(transpose([1 1 1 1 1 1 1 1 1 0]), CYBER_FAULT));
      |
      | Conn_Fault=max([Dos_attack  Mechanical_Fault  1-POWER 1-ROOM_QoS] );
      |
      | %Operative_Level=(1-Conn_Fault)*max(max(TLC_CONN),0.5);
      | Operative_Level=(1-Conn_Fault)*(1-0.5*max(Cyber_Fault))*(1-Service_Fault);
      mask step_sended=|
      | TLC_CONN=Connection*(1-Conn_Fault);
      | TLC_SERVICE=TLC_services*(1-Conn_Fault)+10*TLC_revoke;
      |
      | Cyber_Transmitted=min(Cyber_Fault, transpose([0 0 1 0 1 1 0 0 0 1]));
      | CYBER_FAULT=Cyber_Transmitted*(1-Conn_Fault);
      |
      | ROUTING_QoS=Operative_Level;
      mask prompts: Parameter1 "entity name"; Parameter2 "sampling time"; Parameter3 "project"; resources "input resources and state variables"; Parameter10 "Bring state variables to output"; codeupdate "update code from mask"
      mask help: This is a level-2 MATLAB file S-function which demonstrates CISIA entity
      mask DialogControl Container1 Prompt: All parameters
      mask Display: disp('HuaweiSwitch')
  Heating_Coil (123) : M-S-Function  FunctionName=cisia_msfun  Parameters=Parameter1, Parameter2, Parameter3, resources, Parameter10, codeupdate, step_received, step_computed, dynamic_computed, step_sended, id_entity, id_project, id_type, name_type, color  mask(S-function:msfcn_unit_delay){Parameter1='Heating_Coil', Parameter2=1, Parameter3='ORO', resources=, Parameter10=off, codeupdate=off, step_received=|, step_computed=, dynamic_computed=, step_sended=AIR=Operative_Level;, id_entity=123, id_project=6, id_type=35, name_type=Air_Conditioning_Element, color=#79DE31}
      mask step_received=|
      | Power_Fault=1-POWER;
      | Air_Fault=1-AIR;
      |
      | Operative_Level=min([1-Mechanical_Fault 1-Power_Fault 1-Air_Fault]);
      mask prompts: Parameter1 "entity name"; Parameter2 "sampling time"; Parameter3 "project"; resources "input resources and state variables"; Parameter10 "Bring state variables to output"; codeupdate "update code from mask"
      mask help: This is a level-2 MATLAB file S-function which demonstrates CISIA entity
      mask DialogControl Container1 Prompt: All parameters
      mask Display: disp('Air_Conditioning_Element')
  House_1 (145) : M-S-Function  FunctionName=cisia_msfun  Parameters=Parameter1, Parameter2, Parameter3, resources, Parameter10, codeupdate, step_received, step_computed, dynamic_computed, step_sended, id_entity, id_project, id_type, name_type, color  mask(S-function:msfcn_unit_delay){Parameter1='House_1', Parameter2=1, Parameter3='ORO', resources=, Parameter10=off, codeupdate=off, step_received=|, step_computed=, dynamic_computed=, step_sended=|, id_entity=145, id_project=6, id_type=37, name_type=House, color=#D95319}
      mask step_received=|
      | Connection=max(Connection_init,NGPON_CONN);
      | TLC_services=max(TLC_services_init,TLC_SERVICE);
      | TLC_services=mod(TLC_services,10);
      | TLC_revoke=floor(TLC_SERVICE/10);
      |
      | Cyber_Fault=max(CYBER_FAULT, transpose([Dos_attack   MITM_attack Virus_Attack Port_Scan_Attack  BGP_hijacking BotNet_Attack Data_Corruption SW_Change Config_Change Port_Saturation]));
      |
      | % Vale 1 in presenza di fault
      | Conn_Fault=max([Dos_attack  Mechanical_Fault  1-POWER] );
      |
      | Service_Fault=max(abs(Consumed_Services.*TLC_services-Consumed_Services));
      | Redundancy_Fault=max(abs(Consumed_Services.*NGPON_CONN-Consumed_Services));
      |
      | Alt_Serv_Fault=max(abs(Alternative_Services.*NGPON_CONN-Alternative_Services));
      |
      | Alt_Rout_Fault=max(abs(Consumed_Services.*NGPON_CONN-Consumed_Services));
      |
      | Port_Isolation=min(max(transpose([1 1 1 1 1 1 1 1 1 0]), CYBER_FAULT));
      |
      |
      | Operative_Level=(1-Conn_Fault)*max(max(NGPON_CONN),0.5)*(((1-Service_Fault)+(1-Redundancy_Fault)+(1-Port_Isolation))/3);
      |
      | Alt_Port_Isol=(1-Conn_Fault)*max(max(NGPON_CONN),0.5)*(((1-Service_Fault)+(1-Redundancy_Fault))/2);
      |
      |
      | % Il servizio utilizzato
      | My_Service=max([(1-Service_Fault) (1-Redundancy_Fault)/2]);
      mask step_sended=|
      | HOME_QoS=My_Service;
      |
      | ALT_SERVICES=1-Alt_Serv_Fault;
      |
      | ALT_ROUTING=1-Alt_Rout_Fault;
      |
      | ALT_PORT_ISOLATION=Alt_Port_Isol;
      mask prompts: Parameter1 "entity name"; Parameter2 "sampling time"; Parameter3 "project"; resources "input resources and state variables"; Parameter10 "Bring state variables to output"; codeupdate "update code from mask"
      mask help: This is a level-2 MATLAB file S-function which demonstrates CISIA entity
      mask DialogControl Container1 Prompt: All parameters
      mask Display: image('Icons/House.png')
  IoT_Gateway_1 (275) : M-S-Function  FunctionName=cisia_msfun  Parameters=Parameter1, Parameter2, Parameter3, resources, Parameter10, codeupdate, step_received, step_computed, dynamic_computed, step_sended, id_entity, id_project, id_type, name_type, color  mask(S-function:msfcn_unit_delay){Parameter1='IoT_Gateway_1', Parameter2=1, Parameter3='ORO', resources=, Parameter10=off, codeupdate=off, step_received=|, step_computed=, dynamic_computed=, step_sended=|, id_entity=275, id_project=6, id_type=60, name_type=IoT_Gateway, color=#FFFFFF}
      mask step_received=|
      | Connection=max(Connection_init,TLC_CONN);
      | TLC_services=max(TLC_services_init,TLC_SERVICE);
      | TLC_services=mod(TLC_services,10);
      | TLC_revoke=floor(TLC_SERVICE/10);
      |
      | Cyber_Fault=max(CYBER_FAULT, transpose([Dos_attack   MITM_attack Virus_Attack Port_Scan_Attack  BGP_hijacking BotNet_Attack Data_Corruption SW_Change Config_Change Port_Saturation]));
      |
      | Conn_Fault=max([Dos_attack BGP_hijacking Route_Poisoning Mechanical_Fault] );
      |
      |
      | Operative_Level=(1-Conn_Fault)*max(max(TLC_services),0.5)*(1-0.5*max(Cyber_Fault));
      mask step_sended=|
      | TLC_CONN=Connection*(1-Conn_Fault);
      | TLC_SERVICE=TLC_services*(1-Conn_Fault)*(1-syslog_adm_login)+10*TLC_revoke;
      |
      | Cyber_Transmitted=min(Cyber_Fault, transpose([0 0 1 0 1 1 0 0 0 1]));
      | CYBER_FAULT=Cyber_Transmitted*(1-Conn_Fault);
      |
      |
      | ROUTING_QoS=Operative_Level;
      mask prompts: Parameter1 "entity name"; Parameter2 "sampling time"; Parameter3 "project"; resources "input resources and state variables"; Parameter10 "Bring state variables to output"; codeupdate "update code from mask"
      mask help: This is a level-2 MATLAB file S-function which demonstrates CISIA entity
      mask DialogControl Container1 Prompt: All parameters
      mask Display: image('Icons/IoT_Gateway.png')
  IoT_Sensor_1 (278) : M-S-Function  FunctionName=cisia_msfun  Parameters=Parameter1, Parameter2, Parameter3, resources, Parameter10, codeupdate, step_received, step_computed, dynamic_computed, step_sended, id_entity, id_project, id_type, name_type, color  mask(S-function:msfcn_unit_delay){Parameter1='IoT_Sensor_1', Parameter2=1, Parameter3='ORO', resources=, Parameter10=off, codeupdate=off, step_received=, step_computed=, dynamic_computed=, step_sended=, id_entity=278, id_project=6, id_type=62, name_type=IoT_Sensor, color=#FFFFFF}
      mask prompts: Parameter1 "entity name"; Parameter2 "sampling time"; Parameter3 "project"; resources "input resources and state variables"; Parameter10 "Bring state variables to output"; codeupdate "update code from mask"
      mask help: This is a level-2 MATLAB file S-function which demonstrates CISIA entity
      mask DialogControl Container1 Prompt: All parameters
      mask Display: disp('IoT_Sensor')
  L2S_1 (226) : M-S-Function  FunctionName=cisia_msfun  Parameters=Parameter1, Parameter2, Parameter3, resources, Parameter10, codeupdate, step_received, step_computed, dynamic_computed, step_sended, id_entity, id_project, id_type, name_type, color  mask(S-function:msfcn_unit_delay){Parameter1='L2S_1', Parameter2=1, Parameter3='ORO', resources=, Parameter10=off, codeupdate=off, step_received=|, step_computed=, dynamic_computed=, step_sended=|, id_entity=226, id_project=6, id_type=24, name_type=Layer2Switch, color=#FFFFFF}
      mask step_received=|
      | Connection=max(Connection_init,TLC_CONN);
      | TLC_services=max(TLC_services_init,TLC_SERVICE);
      | TLC_services=mod(TLC_services,10);
      | TLC_revoke=floor(TLC_SERVICE/10);
      |
      | Cyber_Fault=max(CYBER_FAULT, transpose([Dos_attack   MITM_attack Virus_Attack Port_Scan_Attack  BGP_hijacking BotNet_Attack Data_Corruption SW_Change Config_Change Port_Saturation]));
      |
      | Conn_Fault=max([Dos_attack  Mechanical_Fault  1-POWER 1-ROOM_QoS] );
      |
      | Service_Fault=max(abs(Consumed_Services.*TLC_services-Consumed_Services));
      | Redundancy_Fault=max(abs(Consumed_Services.*TLC_CONN-Consumed_Services));
      |
      | Operative_Level=(1-Conn_Fault)*(1-0.5*max(Cyber_Fault))*(1-Service_Fault)*max(max(TLC_CONN),0.5);
      mask step_sended=|
      | TLC_CONN=Connection*(1-Conn_Fault);
      | TLC_SERVICE=TLC_services*(1-Conn_Fault)*(1-Service_Fault)+10*TLC_revoke;
      |
      | Cyber_Transmitted=min(Cyber_Fault, transpose([0 0 1 0 1 1 0 0 0 1]));
      | CYBER_FAULT=Cyber_Transmitted*(1-Conn_Fault);
      mask prompts: Parameter1 "entity name"; Parameter2 "sampling time"; Parameter3 "project"; resources "input resources and state variables"; Parameter10 "Bring state variables to output"; codeupdate "update code from mask"
      mask help: This is a level-2 MATLAB file S-function which demonstrates CISIA entity
      mask DialogControl Container1 Prompt: All parameters
      mask Display: image('Icons/Layer2Switch.png')
  LocalCloud (261) : M-S-Function  FunctionName=cisia_msfun  Parameters=Parameter1, Parameter2, Parameter3, resources, Parameter10, codeupdate, step_received, step_computed, dynamic_computed, step_sended, id_entity, id_project, id_type, name_type, color  mask(S-function:msfcn_unit_delay){Parameter1='LocalCloud', Parameter2=1, Parameter3='ORO', resources=, Parameter10=off, codeupdate=off, step_received=|, step_computed=, dynamic_computed=, step_sended=|, id_entity=261, id_project=6, id_type=53, name_type=CloudServer, color=#FFFFFF}
      mask step_received=|
      | Connection=max(Connection_init,TLC_CONN);
      | TLC_services=max(TLC_services_init,TLC_SERVICE);
      | TLC_services=mod(TLC_services,10);
      | TLC_revoke=floor(TLC_SERVICE/10);
      |
      | %TLC_services=max(TLC_services_init*(1+cisia.major_time),TLC_SERVICE);
      |
      |
      | Mechanical_Fault=max([Mechanical_Fault Mechanical_Fault_init]);
      |
      | Cyber_Fault=max(CYBER_FAULT, transpose([Dos_attack   MITM_attack Virus_Attack Port_Scan_Attack  BGP_hijacking BotNet_Attack Data_Corruption SW_Change Config_Change Port_Saturation]));
      |
      | Conn_Fault=max([Dos_attack  Mechanical_Fault  1-POWER 1-ROOM_QoS] );
      |
      | Service_Fault=max(abs(Consumed_Services.*TLC_services-Consumed_Services));
      | Redundancy_Fault=max(abs(Consumed_Services.*TLC_CONN-Consumed_Services));
      |
      | Operative_Level=(1-Conn_Fault)*(1-0.5*max(Cyber_Fault))*(1-Service_Fault)*max(max(TLC_CONN),0.5);
      mask step_sended=|
      | TLC_CONN=Connection*(1-Conn_Fault);
      | TLC_SERVICE=TLC_services*(1-Conn_Fault)*(1-Service_Fault)+10*TLC_revoke;
      | CYBER_FAULT=Cyber_Fault*(1-Conn_Fault);
      mask prompts: Parameter1 "entity name"; Parameter2 "sampling time"; Parameter3 "project"; resources "input resources and state variables"; Parameter10 "Bring state variables to output"; codeupdate "update code from mask"
      mask help: This is a level-2 MATLAB file S-function which demonstrates CISIA entity
      mask DialogControl Container1 Prompt: All parameters
      mask Display: image('Icons/CloudServer.png')
  MA5603 (95) : M-S-Function  FunctionName=cisia_msfun  Parameters=Parameter1, Parameter2, Parameter3, resources, Parameter10, codeupdate, step_received, step_computed, dynamic_computed, step_sended, id_entity, id_project, id_type, name_type, color  mask(S-function:msfcn_unit_delay){Parameter1='MA5603', Parameter2=1, Parameter3='ORO', resources=, Parameter10=off, codeupdate=off, step_received=|, step_computed=, dynamic_computed=, step_sended=|, id_entity=95, id_project=6, id_type=20, name_type=DSLAM, color=#C9ABDB}
      mask step_received=|
      | Connection=max(Connection_init,TLC_CONN);
      | TLC_services=max(TLC_services_init,TLC_SERVICE);
      | TLC_services=mod(TLC_services,10);
      | TLC_revoke=floor(TLC_SERVICE/10);
      |
      | Cyber_Fault=max(CYBER_FAULT, transpose([Dos_attack   MITM_attack Virus_Attack Port_Scan_Attack  BGP_hijacking BotNet_Attack Data_Corruption SW_Change Config_Change Port_Saturation]));
      |
      | Port_Isolation=min(max(transpose([1 1 1 1 1 1 1 1 1 0]), CYBER_FAULT));
      |
      |
      | Conn_Fault=max([Dos_attack  Mechanical_Fault  1-POWER] );
      |
      | %Operative_Level=(1-Conn_Fault)*max(max(TLC_services),0.5);
      |
      | Operative_Level=(1-Conn_Fault)*(1-0.5*max(Cyber_Fault))*max(max(TLC_services),0.5);
      mask step_sended=|
      | TLC_CONN=Connection*(1-Conn_Fault);
      | TLC_SERVICE=TLC_services*(1-Conn_Fault)+10*TLC_revoke;
      |
      | ADSL_CONN=Connection*(1-Conn_Fault);
      | ADSL_QoS=Operative_Level;
      |
      | Cyber_Transmitted=min(Cyber_Fault, transpose([0 0 1 0 1 1 0 0 0 1]));
      | CYBER_FAULT=Cyber_Transmitted*(1-Conn_Fault);
      mask prompts: Parameter1 "entity name"; Parameter2 "sampling time"; Parameter3 "project"; resources "input resources and state variables"; Parameter10 "Bring state variables to output"; codeupdate "update code from mask"
      mask help: This is a level-2 MATLAB file S-function which demonstrates CISIA entity
      mask DialogControl Container1 Prompt: All parameters
      mask Display: image('Icons/MA5603.png')
  Medical_6 (176) : M-S-Function  FunctionName=cisia_msfun  Parameters=Parameter1, Parameter2, Parameter3, resources, Parameter10, codeupdate, step_received, step_computed, dynamic_computed, step_sended, id_entity, id_project, id_type, name_type, color  mask(S-function:msfcn_unit_delay){Parameter1='Medical_6', Parameter2=1, Parameter3='ORO', resources=, Parameter10=off, codeupdate=off, step_received=|, step_computed=, dynamic_computed=, step_sended=|, id_entity=176, id_project=6, id_type=25, name_type=Medical_Room, color=#00FFFF}
      mask step_received=|
      | Connection=max(Connection_init,TLC_CONN);
      | TLC_services=max(TLC_services_init,TLC_SERVICE);
      | TLC_services=mod(TLC_services,10);
      | TLC_revoke=floor(TLC_SERVICE/10);
      |
      | Conn_Fault=max([Power_Fault 1-POWER 1-MOBILE_QoS]);
      |
      | Water_Fault=1-WATER;
      | Air_Fault=1-AIR;
      | Physical_Fault=max([Water_Fault Air_Fault 1-OXYGEN]);
      |
      | Alt_Serv_Fault=max(abs(Alternative_Services.*TLC_CONN-Alternative_Services));
      |
      | Alt_Rout_Fault=max(abs(Consumed_Services.*TLC_CONN-Consumed_Services));
      |
      |
      | Service_Fault=max(abs(Consumed_Services.*TLC_services-Consumed_Services));
      | Redundancy_Fault=max(abs(Consumed_Services.*TLC_CONN-Consumed_Services));
      |
      | Operative_Level=(1-Conn_Fault)*(1-0.5*Physical_Fault)*(1-0.5*Service_Fault);
      mask step_sended=|
      | MEDICAL_ROOM_QoS=Operative_Level;
      |
      | ALT_SERVICES=1-Alt_Serv_Fault;
      | ALT_ROUTING=1-Alt_Rout_Fault;
      mask prompts: Parameter1 "entity name"; Parameter2 "sampling time"; Parameter3 "project"; resources "input resources and state variables"; Parameter10 "Bring state variables to output"; codeupdate "update code from mask"
      mask help: This is a level-2 MATLAB file S-function which demonstrates CISIA entity
      mask DialogControl Container1 Prompt: All parameters
      mask Display: disp('Medical_Room')
  Mobile_1 (147) : M-S-Function  FunctionName=cisia_msfun  Parameters=Parameter1, Parameter2, Parameter3, resources, Parameter10, codeupdate, step_received, step_computed, dynamic_computed, step_sended, id_entity, id_project, id_type, name_type, color  mask(S-function:msfcn_unit_delay){Parameter1='Mobile_1', Parameter2=1, Parameter3='ORO', resources=, Parameter10=off, codeupdate=off, step_received=|, step_computed=, dynamic_computed=, step_sended=|, id_entity=147, id_project=6, id_type=39, name_type=MobileUnit, color=#C9ABDB}
      mask step_received=|
      | Connection=max(Connection_init,R_CONN);
      | TLC_services=max(TLC_services_init,TLC_SERVICE);
      | TLC_services=mod(TLC_services,10);
      | TLC_revoke=floor(TLC_SERVICE/10);
      |
      | Service_Fault=max(abs(Consumed_Services.*TLC_services-Consumed_Services));
      | Redundancy_Fault=max(abs(Consumed_Services.*R_CONN-Consumed_Services));
      |
      | Alt_Serv_Fault=max(abs(Alternative_Services.*R_CONN-Alternative_Services));
      |
      | Alt_Rout_Fault=max(abs(Consumed_Services.*R_CONN-Consumed_Services));
      |
      | Port_Isolation=min(max(transpose([1 1 1 1 1 1 1 1 1 0]), CYBER_FAULT));
      |
      |
      | Operative_Level=(1-Mechanical_Fault)*max(max(R_CONN), 0.5)*(((1-Service_Fault)+(1-Redundancy_Fault)+(1-Port_Isolation))/3);
      |
      | Alt_Port_Isol=(1-Mechanical_Fault)*max(max(R_CONN), 0.5)*(((1-Service_Fault)+(1-Redundancy_Fault))/2);
      mask step_sended=|
      | MOBILE_QoS=Operative_Level;
      |
      |
      | ALT_SERVICES=1-Alt_Serv_Fault;
      | ALT_ROUTING=1-Alt_Rout_Fault;
      | ALT_PORT_ISOLATION=Alt_Port_Isol;
      mask prompts: Parameter1 "entity name"; Parameter2 "sampling time"; Parameter3 "project"; resources "input resources and state variables"; Parameter10 "Bring state variables to output"; codeupdate "update code from mask"
      mask help: This is a level-2 MATLAB file S-function which demonstrates CISIA entity
      mask DialogControl Container1 Prompt: All parameters
      mask Display: image('Icons/MobileUnit.png')
  Mobile_2 (148) : M-S-Function  FunctionName=cisia_msfun  Parameters=Parameter1, Parameter2, Parameter3, resources, Parameter10, codeupdate, step_received, step_computed, dynamic_computed, step_sended, id_entity, id_project, id_type, name_type, color  mask(S-function:msfcn_unit_delay){Parameter1='Mobile_2', Parameter2=1, Parameter3='ORO', resources=, Parameter10=off, codeupdate=off, step_received=|, step_computed=, dynamic_computed=, step_sended=|, id_entity=148, id_project=6, id_type=39, name_type=MobileUnit, color=#C9ABDB}
      mask step_received=|
      | Connection=max(Connection_init,R_CONN);
      | TLC_services=max(TLC_services_init,TLC_SERVICE);
      | TLC_services=mod(TLC_services,10);
      | TLC_revoke=floor(TLC_SERVICE/10);
      |
      | Service_Fault=max(abs(Consumed_Services.*TLC_services-Consumed_Services));
      | Redundancy_Fault=max(abs(Consumed_Services.*R_CONN-Consumed_Services));
      |
      | Alt_Serv_Fault=max(abs(Alternative_Services.*R_CONN-Alternative_Services));
      |
      | Alt_Rout_Fault=max(abs(Consumed_Services.*R_CONN-Consumed_Services));
      |
      | Port_Isolation=min(max(transpose([1 1 1 1 1 1 1 1 1 0]), CYBER_FAULT));
      |
      |
      | Operative_Level=(1-Mechanical_Fault)*max(max(R_CONN), 0.5)*(((1-Service_Fault)+(1-Redundancy_Fault)+(1-Port_Isolation))/3);
      |
      | Alt_Port_Isol=(1-Mechanical_Fault)*max(max(R_CONN), 0.5)*(((1-Service_Fault)+(1-Redundancy_Fault))/2);
      mask step_sended=|
      | MOBILE_QoS=Operative_Level;
      |
      |
      | ALT_SERVICES=1-Alt_Serv_Fault;
      | ALT_ROUTING=1-Alt_Rout_Fault;
      | ALT_PORT_ISOLATION=Alt_Port_Isol;
      mask prompts: Parameter1 "entity name"; Parameter2 "sampling time"; Parameter3 "project"; resources "input resources and state variables"; Parameter10 "Bring state variables to output"; codeupdate "update code from mask"
      mask help: This is a level-2 MATLAB file S-function which demonstrates CISIA entity
      mask DialogControl Container1 Prompt: All parameters
      mask Display: image('Icons/MobileUnit.png')
  NOC (272) : M-S-Function  FunctionName=cisia_msfun  Parameters=Parameter1, Parameter2, Parameter3, resources, Parameter10, codeupdate, step_received, step_computed, dynamic_computed, step_sended, id_entity, id_project, id_type, name_type, color  mask(S-function:msfcn_unit_delay){Parameter1='NOC', Parameter2=1, Parameter3='ORO', resources=, Parameter10=off, codeupdate=off, step_received=|, step_computed=, dynamic_computed=, step_sended=WORKSTATION_QoS=Operative_Level;, id_entity=272, id_project=6, id_type=43, name_type=Workstation, color=#FFFFFF}
      mask step_received=|
      | Connection=max(Connection_init,TLC_CONN);
      |
      | Cyber_Fault=max(CYBER_FAULT, transpose([Dos_attack   MITM_attack Virus_Attack Port_Scan_Attack  BGP_hijacking BotNet_Attack Data_Corruption SW_Change Config_Change Port_Saturation]));
      |
      | % Vale 1 in presenza di fault
      | Conn_Fault=max([Dos_attack  Mechanical_Fault  1-POWER] );
      |
      |
      |
      | Operative_Level=(1-Conn_Fault)*max(max(TLC_CONN),0.5);
      mask prompts: Parameter1 "entity name"; Parameter2 "sampling time"; Parameter3 "project"; resources "input resources and state variables"; Parameter10 "Bring state variables to output"; codeupdate "update code from mask"
      mask help: This is a level-2 MATLAB file S-function which demonstrates CISIA entity
      mask DialogControl Container1 Prompt: All parameters
      mask Display: image('Icons/Workstation.png')
  Nex_1 (3) : M-S-Function  FunctionName=cisia_msfun  Parameters=Parameter1, Parameter2, Parameter3, resources, Parameter10, codeupdate, step_received, step_computed, dynamic_computed, step_sended, id_entity, id_project, id_type, name_type, color  mask(S-function:msfcn_unit_delay){Parameter1='Nex_1', Parameter2=1, Parameter3='ORO', resources=, Parameter10=off, codeupdate=off, step_received=|, step_computed=, dynamic_computed=, step_sended=|, id_entity=3, id_project=6, id_type=2, name_type=Nexus93180Switch, color=#0072BD}
      mask step_received=|
      | Connection=max(Connection_init,TLC_CONN);
      |
      | TLC_services=max(TLC_services_init,TLC_SERVICE);
      | TLC_services=mod(TLC_services,10);
      | TLC_revoke=floor(TLC_SERVICE/10);
      |
      | Cyber_Fault=max(CYBER_FAULT, transpose([Dos_attack   MITM_attack Virus_Attack Port_Scan_Attack  BGP_hijacking BotNet_Attack Data_Corruption SW_Change Config_Change Port_Saturation]));
      |
      | Conn_Fault=max([Dos_attack  Mechanical_Fault  1-POWER 1-ROOM_QoS] );
      |
      | Operative_Level=(1-Conn_Fault)*max(max(TLC_services),0.5)*(1-0.5*max(Cyber_Fault));
      mask step_sended=|
      | TLC_CONN=Connection*(1-Conn_Fault);
      | TLC_SERVICE=TLC_services*(1-Conn_Fault)+10*TLC_revoke;
      |
      | Cyber_Transmitted=min(Cyber_Fault, transpose([0 0 1 0 1 1 0 0 0 1]));
      | CYBER_FAULT=Cyber_Transmitted*(1-Conn_Fault);
      |
      |
      | SWITCHING_QoS=Operative_Level;
      mask prompts: Parameter1 "entity name"; Parameter2 "sampling time"; Parameter3 "project"; resources "input resources and state variables"; Parameter10 "Bring state variables to output"; codeupdate "update code from mask"
      mask help: This is a level-2 MATLAB file S-function which demonstrates CISIA entity
      mask DialogControl Container1 Prompt: All parameters
      mask Display: image('Icons/Nexus93180Switch.png')
  OLT_1 (25) : M-S-Function  FunctionName=cisia_msfun  Parameters=Parameter1, Parameter2, Parameter3, resources, Parameter10, codeupdate, step_received, step_computed, dynamic_computed, step_sended, id_entity, id_project, id_type, name_type, color  mask(S-function:msfcn_unit_delay){Parameter1='OLT_1', Parameter2=1, Parameter3='ORO', resources=, Parameter10=off, codeupdate=off, step_received=|, step_computed=, dynamic_computed=, step_sended=|, id_entity=25, id_project=6, id_type=4, name_type=OLT, color=#FF6929}
      mask step_received=|
      | Connection=max(Connection_init,TLC_CONN);
      | TLC_services=max(TLC_services_init,TLC_SERVICE);
      | TLC_services=mod(TLC_services,10);
      | TLC_revoke=floor(TLC_SERVICE/10);
      |
      | Cyber_Fault=max(CYBER_FAULT, transpose([Dos_attack   MITM_attack Virus_Attack Port_Scan_Attack  BGP_hijacking BotNet_Attack Data_Corruption SW_Change Config_Change Port_Saturation]));
      |
      |
      | % Vale 1 in presenza di fault
      | Conn_Fault=max([Dos_attack  Mechanical_Fault  1-POWER 1-ROOM_QoS] );
      |
      |
      | Service_Fault=max(abs(Consumed_Services.*TLC_services-Consumed_Services));
      |
      |
      | Redundancy_Fault=max(abs(Consumed_Services.*TLC_CONN-Consumed_Services));
      |
      | Operative_Level=(1-Conn_Fault)*(1-0.5*max(Cyber_Fault))*(1-Service_Fault)*max(max(TLC_CONN),0.5);
      |
      |
      | %Operative_Level=(1-Conn_Fault)*max(max(TLC_CONN),0.5)*((2*(1-Service_Fault)+(1-Redundancy_Fault))/3);
      | %My_Service=max([(1-Service_Fault) (1-Redundancy_Fault)/2]);
      | %Operative_Level=(1-Conn_Fault)*My_Service;
      mask step_sended=|
      | TLC_CONN=Connection*(1-Conn_Fault);
      | TLC_SERVICE=TLC_services*(1-Conn_Fault)+10*TLC_revoke;
      |
      | Cyber_Transmitted=min(Cyber_Fault, transpose([0 0 1 0 1 1 0 0 0 1]));
      | CYBER_FAULT=Cyber_Transmitted*(1-Conn_Fault);
      |
      | NGPON_CONN=TLC_CONN;
      mask prompts: Parameter1 "entity name"; Parameter2 "sampling time"; Parameter3 "project"; resources "input resources and state variables"; Parameter10 "Bring state variables to output"; codeupdate "update code from mask"
      mask help: This is a level-2 MATLAB file S-function which demonstrates CISIA entity
      mask DialogControl Container1 Prompt: All parameters
      mask Display: disp('OLT')
  ONU_2 (58) : M-S-Function  FunctionName=cisia_msfun  Parameters=Parameter1, Parameter2, Parameter3, resources, Parameter10, codeupdate, step_received, step_computed, dynamic_computed, step_sended, id_entity, id_project, id_type, name_type, color  mask(S-function:msfcn_unit_delay){Parameter1='ONU_2', Parameter2=1, Parameter3='ORO', resources=, Parameter10=off, codeupdate=off, step_received=|, step_computed=, dynamic_computed=, step_sended=|, id_entity=58, id_project=6, id_type=12, name_type=ONU, color=#90DB5A}
      mask step_received=|
      | Connection=max(Connection_init,NGPON_CONN);
      | TLC_services=max(TLC_services_init,TLC_SERVICE);
      | TLC_services=mod(TLC_services,10);
      | TLC_revoke=floor(TLC_SERVICE/10);
      |
      | Cyber_Fault=max(CYBER_FAULT, transpose([Dos_attack   MITM_attack Virus_Attack Port_Scan_Attack  BGP_hijacking BotNet_Attack Data_Corruption SW_Change Config_Change Port_Saturation]));
      |
      | Conn_Fault=max([Dos_attack  Mechanical_Fault  1-POWER] );
      |
      | Service_Fault=max(abs(Consumed_Services.*TLC_services-Consumed_Services));
      | Redundancy_Fault=max(abs(Consumed_Services.*NGPON_CONN-Consumed_Services));
      |
      | Operative_Level=(1-Conn_Fault)*(1-0.5*max(Cyber_Fault))*(1-Service_Fault)*max(max(NGPON_CONN),0.5);
      |
      | %Operative_Level=(1-Conn_Fault)*max(max(TLC_services),0.5)*((2*(1-Service_Fault)+(1-Redundancy_Fault))/3);
      | % Il servizio utilizzato
      | %My_Service=max([(1-Service_Fault) (1-Redundancy_Fault)/2]);
      | %Operative_Level=(1-Conn_Fault);
      mask step_sended=|
      | TLC_SERVICE=TLC_services*(1-Conn_Fault)+10*TLC_revoke;
      | NGPON_CONN=Connection*(1-Conn_Fault);
      |
      | Cyber_Transmitted=min(Cyber_Fault, transpose([0 0 1 0 1 1 0 0 0 1]));
      | CYBER_FAULT=Cyber_Transmitted*(1-Conn_Fault);
      mask prompts: Parameter1 "entity name"; Parameter2 "sampling time"; Parameter3 "project"; resources "input resources and state variables"; Parameter10 "Bring state variables to output"; codeupdate "update code from mask"
      mask help: This is a level-2 MATLAB file S-function which demonstrates CISIA entity
      mask DialogControl Container1 Prompt: All parameters
      mask Display: disp('ONU')
  Oxygen_Duct_1 (263) : M-S-Function  FunctionName=cisia_msfun  Parameters=Parameter1, Parameter2, Parameter3, resources, Parameter10, codeupdate, step_received, step_computed, dynamic_computed, step_sended, id_entity, id_project, id_type, name_type, color  mask(S-function:msfcn_unit_delay){Parameter1='Oxygen_Duct_1', Parameter2=1, Parameter3='ORO', resources=, Parameter10=off, codeupdate=off, step_received=Operative_Level=(1-Mechanical_Fault)*(1-0.5*(1-OXYGEN));, step_computed=, dynamic_computed=, step_sended=OXYGEN=Operative_Level;, id_entity=263, id_project=6, id_type=57, name_type=OXYGEN_Duct, color=#E85151}
      mask prompts: Parameter1 "entity name"; Parameter2 "sampling time"; Parameter3 "project"; resources "input resources and state variables"; Parameter10 "Bring state variables to output"; codeupdate "update code from mask"
      mask help: This is a level-2 MATLAB file S-function which demonstrates CISIA entity
      mask DialogControl Container1 Prompt: All parameters
      mask Display: disp('OXYGEN_Duct')
  Physical_Access_Server_1 (158) : M-S-Function  FunctionName=cisia_msfun  Parameters=Parameter1, Parameter2, Parameter3, resources, Parameter10, codeupdate, step_received, step_computed, dynamic_computed, step_sended, id_entity, id_project, id_type, name_type, color  mask(S-function:msfcn_unit_delay){Parameter1='Physical_Access_Server_1', Parameter2=1, Parameter3='ORO', resources=, Parameter10=off, codeupdate=off, step_received=|, step_computed=, dynamic_computed=, step_sended=|, id_entity=158, id_project=6, id_type=40, name_type=App_Server, color=#00AAFF}
      mask step_received=|
      | Connection=max(Connection_init,TLC_CONN);
      | TLC_services=max(TLC_services_init,TLC_SERVICE);
      | TLC_services=mod(TLC_services,10);
      | TLC_revoke=floor(TLC_SERVICE/10);
      |
      | Mechanical_Fault=max([Mechanical_Fault Mechanical_Fault_init]);
      |
      | %if strcmp(name_entity,"BlockChainServer") && (cisia.major_time>=2)
      |  % Dos_attack=1;
      |  %TLC_revoke(9)=1;
      |  %TLC_services(9)=0;
      | %end
      |
      |
      | Cyber_Fault=max(CYBER_FAULT, transpose([Dos_attack   MITM_attack Virus_Attack Port_Scan_Attack  BGP_hijacking BotNet_Attack Data_Corruption SW_Change Config_Change Port_Saturation]));
      |
      | Service_Fault=max(abs(Consumed_Services.*TLC_services-Consumed_Services));
      | Redundancy_Fault=max(abs(Consumed_Services.*TLC_CONN-Consumed_Services));
      |
      | Conn_Fault=max([Dos_attack  Mechanical_Fault  1-POWER 1-ROOM_QoS] );
      |
      |
      | Operative_Level=(1-Conn_Fault)*(1-0.5*max(Cyber_Fault))*(1-Service_Fault)*max(max(TLC_CONN),0.5);
      mask step_sended=|
      | TLC_CONN=Connection*(1-Conn_Fault);
      | TLC_SERVICE=TLC_services*(1-Conn_Fault)*(1-Service_Fault)*(1-syslog_adm_login)+10*TLC_revoke;
      | CYBER_FAULT=Cyber_Fault*(1-Conn_Fault);
      mask prompts: Parameter1 "entity name"; Parameter2 "sampling time"; Parameter3 "project"; resources "input resources and state variables"; Parameter10 "Bring state variables to output"; codeupdate "update code from mask"
      mask help: This is a level-2 MATLAB file S-function which demonstrates CISIA entity
      mask DialogControl Container1 Prompt: All parameters
      mask Display: image('Icons/App_Server.png')
  Pipe_1 (120) : M-S-Function  FunctionName=cisia_msfun  Parameters=Parameter1, Parameter2, Parameter3, resources, Parameter10, codeupdate, step_received, step_computed, dynamic_computed, step_sended, id_entity, id_project, id_type, name_type, color  mask(S-function:msfcn_unit_delay){Parameter1='Pipe_1', Parameter2=1, Parameter3='ORO', resources=, Parameter10=off, codeupdate=off, step_received=|, step_computed=, dynamic_computed=, step_sended=|, id_entity=120, id_project=6, id_type=32, name_type=Pipe, color=#78C6FA}
      mask step_received=|
      | Water_Fault= 1- WATER;
      | Operative_Level=(1-Mechanical_Fault)*(1-0.5*Water_Fault);
      mask step_sended=|
      | WATER=Operative_Level;
      | PIPE_QoS=Operative_Level;
      mask prompts: Parameter1 "entity name"; Parameter2 "sampling time"; Parameter3 "project"; resources "input resources and state variables"; Parameter10 "Bring state variables to output"; codeupdate "update code from mask"
      mask help: This is a level-2 MATLAB file S-function which demonstrates CISIA entity
      mask DialogControl Container1 Prompt: All parameters
      mask Display: disp('Pipe')
  PowerGen_3 (157) : M-S-Function  FunctionName=cisia_msfun  Parameters=Parameter1, Parameter2, Parameter3, resources, Parameter10, codeupdate, step_received, step_computed, dynamic_computed, step_sended, id_entity, id_project, id_type, name_type, color  mask(S-function:msfcn_unit_delay){Parameter1='PowerGen_3', Parameter2=1, Parameter3='ORO', resources=, Parameter10=off, codeupdate=off, step_received=Operative_Level=1-Power_Fault;, step_computed=, dynamic_computed=, step_sended=POWER=Operative_Level;, id_entity=157, id_project=6, id_type=8, name_type=PowerSource, color=#84BD8C}
      mask prompts: Parameter1 "entity name"; Parameter2 "sampling time"; Parameter3 "project"; resources "input resources and state variables"; Parameter10 "Bring state variables to output"; codeupdate "update code from mask"
      mask help: This is a level-2 MATLAB file S-function which demonstrates CISIA entity
      mask DialogControl Container1 Prompt: All parameters
      mask Display: image('Icons/PowerSource.png')
  Primary_Cabin_1 (315) : M-S-Function  FunctionName=cisia_msfun  Parameters=Parameter1, Parameter2, Parameter3, resources, Parameter10, codeupdate, step_received, step_computed, dynamic_computed, step_sended, id_entity, id_project, id_type, name_type, color  mask(S-function:msfcn_unit_delay){Parameter1='Primary_Cabin_1', Parameter2=1, Parameter3='ORO', resources=, Parameter10=off, codeupdate=off, step_received=|, step_computed=, dynamic_computed=, step_sended=|, id_entity=315, id_project=6, id_type=66, name_type=Electric_Plant, color=#FFFFFF}
      mask step_received=|
      | Connection=max(Connection_init,TLC_CONN);
      | TLC_services=max(TLC_services_init,TLC_SERVICE);
      | TLC_services=mod(TLC_services,10);
      | TLC_revoke=floor(TLC_SERVICE/10);
      |
      |
      | Physical_Fault=max(Fire_Fault,Mechanical_Fault);
      |
      | Service_Fault=max(abs(Consumed_Services.*TLC_services-Consumed_Services));
      | Redundancy_Fault=max(abs(Consumed_Services.*TLC_CONN-Consumed_Services));
      |
      | Alt_Serv_Fault=max(abs(Alternative_Services.*TLC_CONN-Alternative_Services));
      |
      | Alt_Rout_Fault=max(abs(Consumed_Services.*TLC_CONN-Consumed_Services));
      |
      | Operative_Level=(1-Physical_Fault)*max(max(TLC_CONN), 0.5)*(((1-Service_Fault)+(1-Redundancy_Fault))/2);
      mask step_sended=|
      | E_POWER_1=Power_Gen*Operative_Level;
      |
      |
      | TLC_CONN=Connection*(1-Conn_Fault);
      | TLC_SERVICE=TLC_services*(1-Room_Fault)*(1-Conn_Fault)*(1-syslog_adm_login)+10*TLC_revoke;
      |
      |
      | Cyber_Transmitted=min(Cyber_Fault, transpose([0 0 1 0 1 1 0 0 0 1]));
      |
      | CYBER_FAULT=Cyber_Transmitted*(1-Conn_Fault);
      |
      |
      | PRIMARY_CABIN_QoS=Operative_Level;
      |
      | ALT_SERVICES=1-Alt_Serv_Fault;
      | ALT_ROUTING=1-Alt_Rout_Fault;
      mask prompts: Parameter1 "entity name"; Parameter2 "sampling time"; Parameter3 "project"; resources "input resources and state variables"; Parameter10 "Bring state variables to output"; codeupdate "update code from mask"
      mask help: This is a level-2 MATLAB file S-function which demonstrates CISIA entity
      mask DialogControl Container1 Prompt: All parameters
      mask Display: image('Icons/Primary_Cabin_1.png')
  RADIO_BRIDGE_2 (277) : M-S-Function  FunctionName=cisia_msfun  Parameters=Parameter1, Parameter2, Parameter3, resources, Parameter10, codeupdate, step_received, step_computed, dynamic_computed, step_sended, id_entity, id_project, id_type, name_type, color  mask(S-function:msfcn_unit_delay){Parameter1='RADIO_BRIDGE_2', Parameter2=1, Parameter3='ORO', resources=, Parameter10=off, codeupdate=off, step_received=|, step_computed=, dynamic_computed=, step_sended=|, id_entity=277, id_project=6, id_type=61, name_type=Radio_Bridge, color=#FFFFFF}
      mask step_received=|
      | Connection=TLC_CONN;
      | TLC_services=TLC_SERVICE;
      | Cyber_Fault=CYBER_FAULT;
      mask step_sended=|
      | TLC_CONN=Connection;
      | TLC_SERVICE=TLC_services;
      | CYBER_FAULT=Cyber_Fault;
      mask prompts: Parameter1 "entity name"; Parameter2 "sampling time"; Parameter3 "project"; resources "input resources and state variables"; Parameter10 "Bring state variables to output"; codeupdate "update code from mask"
      mask help: This is a level-2 MATLAB file S-function which demonstrates CISIA entity
      mask DialogControl Container1 Prompt: All parameters
      mask Display: image('Icons/Radio_Bridge.png')
  RECEIVER_1 (273) : M-S-Function  FunctionName=cisia_msfun  Parameters=Parameter1, Parameter2, Parameter3, resources, Parameter10, codeupdate, step_received, step_computed, dynamic_computed, step_sended, id_entity, id_project, id_type, name_type, color  mask(S-function:msfcn_unit_delay){Parameter1='RECEIVER_1', Parameter2=1, Parameter3='ORO', resources=, Parameter10=off, codeupdate=off, step_received=Conn_Fault=1-VDES_CONN;, step_computed=, dynamic_computed=, step_sended=VDES_CONN=1-Conn_Fault;, id_entity=273, id_project=6, id_type=59, name_type=VDES_RECEIVER, color=#FFFFFF}
      mask prompts: Parameter1 "entity name"; Parameter2 "sampling time"; Parameter3 "project"; resources "input resources and state variables"; Parameter10 "Bring state variables to output"; codeupdate "update code from mask"
      mask help: This is a level-2 MATLAB file S-function which demonstrates CISIA entity
      mask DialogControl Container1 Prompt: All parameters
      mask Display: image('Icons/VDES_RECEIVER.png')
  RESISTO_1 (196) : M-S-Function  FunctionName=cisia_msfun  Parameters=Parameter1, Parameter2, Parameter3, resources, Parameter10, codeupdate, step_received, step_computed, dynamic_computed, step_sended, id_entity, id_project, id_type, name_type, color  mask(S-function:msfcn_unit_delay){Parameter1='RESISTO_1', Parameter2=1, Parameter3='ORO', resources=, Parameter10=off, codeupdate=off, step_received=|, step_computed=, dynamic_computed=, step_sended=WORKSTATION_QoS=Operative_Level;, id_entity=196, id_project=6, id_type=43, name_type=Workstation, color=#FFFFFF}
      mask step_received=|
      | Connection=max(Connection_init,TLC_CONN);
      |
      | Cyber_Fault=max(CYBER_FAULT, transpose([Dos_attack   MITM_attack Virus_Attack Port_Scan_Attack  BGP_hijacking BotNet_Attack Data_Corruption SW_Change Config_Change Port_Saturation]));
      |
      | % Vale 1 in presenza di fault
      | Conn_Fault=max([Dos_attack  Mechanical_Fault  1-POWER] );
      |
      |
      |
      | Operative_Level=(1-Conn_Fault)*max(max(TLC_CONN),0.5);
      mask prompts: Parameter1 "entity name"; Parameter2 "sampling time"; Parameter3 "project"; resources "input resources and state variables"; Parameter10 "Bring state variables to output"; codeupdate "update code from mask"
      mask help: This is a level-2 MATLAB file S-function which demonstrates CISIA entity
      mask DialogControl Container1 Prompt: All parameters
      mask Display: image('Icons/RESISTO_1.png')
  Remote_Site (334) : M-S-Function  FunctionName=cisia_msfun  Parameters=Parameter1, Parameter2, Parameter3, resources, Parameter10, codeupdate, step_received, step_computed, dynamic_computed, step_sended, id_entity, id_project, id_type, name_type, color  mask(S-function:msfcn_unit_delay){Parameter1='Remote_Site', Parameter2=1, Parameter3='ORO', resources=, Parameter10=off, codeupdate=off, step_received=|, step_computed=, dynamic_computed=, step_sended=|, id_entity=334, id_project=6, id_type=79, name_type=Site, color=#FFFFFF}
      mask step_received=|
      | Connection=max(Connection_init,TLC_CONN);
      | TLC_services=max(TLC_services_init,TLC_SERVICE);
      | TLC_services=mod(TLC_services,10);
      | TLC_revoke=floor(TLC_SERVICE/10);
      |
      | Service_Fault=max(abs(Consumed_Services.*TLC_services-Consumed_Services));
      | Redundancy_Fault=max(abs(Consumed_Services.*TLC_CONN-Consumed_Services));
      |
      | Alt_Serv_Fault=max(abs(Alternative_Services.*TLC_CONN-Alternative_Services));
      |
      | Alt_Rout_Fault=max(abs(Consumed_Services.*TLC_CONN-Consumed_Services));
      |
      | Operative_Level=(1-Mechanical_Fault)*max(max(TLC_CONN), 0.5)*(((1-Service_Fault)+(1-Redundancy_Fault))/2);
      mask step_sended=|
      | SITE_QoS=Operative_Level;
      |
      | ALT_SERVICES=1-Alt_Serv_Fault;
      | ALT_ROUTING=1-Alt_Rout_Fault;
      mask prompts: Parameter1 "entity name"; Parameter2 "sampling time"; Parameter3 "project"; resources "input resources and state variables"; Parameter10 "Bring state variables to output"; codeupdate "update code from mask"
      mask help: This is a level-2 MATLAB file S-function which demonstrates CISIA entity
      mask DialogControl Container1 Prompt: All parameters
      mask Display: image('Icons/Site.png')
  Robot_1 (203) : M-S-Function  FunctionName=cisia_msfun  Parameters=Parameter1, Parameter2, Parameter3, resources, Parameter10, codeupdate, step_received, step_computed, dynamic_computed, step_sended, id_entity, id_project, id_type, name_type, color  mask(S-function:msfcn_unit_delay){Parameter1='Robot_1', Parameter2=1, Parameter3='ORO', resources=, Parameter10=off, codeupdate=off, step_received=|, step_computed=, dynamic_computed=, step_sended=|, id_entity=203, id_project=6, id_type=44, name_type=Robot, color=#FFFFFF}
      mask step_received=|
      | Connection=max(Connection_init,R_CONN);
      | TLC_services=max(TLC_services_init,TLC_SERVICE);
      | TLC_services=mod(TLC_services,10);
      | TLC_revoke=floor(TLC_SERVICE/10);
      |
      | Physical_Fault=max([Mechanical_Fault  1-POWER] );
      |
      | Service_Fault=max(abs(Consumed_Services.*TLC_services-Consumed_Services));
      | Redundancy_Fault=max(abs(Consumed_Services.*R_CONN-Consumed_Services));
      |
      |
      | Alt_Serv_Fault=max(abs(Alternative_Services.*R_CONN-Alternative_Services));
      |
      | Alt_Rout_Fault=max(abs(Consumed_Services.*R_CONN-Consumed_Services));
      |
      |
      | Operative_Level=(1-Physical_Fault)*max(max(R_CONN),0.5)*(1-0.6*Service_Fault);
      mask step_sended=|
      | ROBOT_QoS=Operative_Level;
      |
      |
      | ALT_SERVICES=1-Alt_Serv_Fault;
      | ALT_ROUTING=1-Alt_Rout_Fault;
      mask prompts: Parameter1 "entity name"; Parameter2 "sampling time"; Parameter3 "project"; resources "input resources and state variables"; Parameter10 "Bring state variables to output"; codeupdate "update code from mask"
      mask help: This is a level-2 MATLAB file S-function which demonstrates CISIA entity
      mask DialogControl Container1 Prompt: All parameters
      mask Display: image('Icons/Robot.png')
  Room_1 (51) : M-S-Function  FunctionName=cisia_msfun  Parameters=Parameter1, Parameter2, Parameter3, resources, Parameter10, codeupdate, step_received, step_computed, dynamic_computed, step_sended, id_entity, id_project, id_type, name_type, color  mask(S-function:msfcn_unit_delay){Parameter1='Room_1', Parameter2=1, Parameter3='ORO', resources=, Parameter10=off, codeupdate=off, step_received=|, step_computed=, dynamic_computed=, step_sended=ROOM_QoS=Operative_Level;, id_entity=51, id_project=6, id_type=9, name_type=Room, color=#EDB120}
      mask step_received=|
      | Physical_Fault=max([Power_Fault Flooding_Fault Fire_Fault Cooling_Fault 1-POWER]);
      |
      |
      | %Operative_Level=min([1-Power_Fault 1-Flooding_Fault  1-Fire_Fault  1-Cooling_Fault  POWER]);
      | %Operative_Level=Operative_Level*max((1-Unauthorized_Access),0.5);
      |
      | Operative_Level=(1-Physical_Fault)*(1-0.5*Unauthorized_Access);
      mask prompts: Parameter1 "entity name"; Parameter2 "sampling time"; Parameter3 "project"; resources "input resources and state variables"; Parameter10 "Bring state variables to output"; codeupdate "update code from mask"
      mask help: This is a level-2 MATLAB file S-function which demonstrates CISIA entity
      mask DialogControl Container1 Prompt: All parameters
      mask Display: image('Icons/Room.png')
  Security_Cameras_Server_1 (159) : M-S-Function  FunctionName=cisia_msfun  Parameters=Parameter1, Parameter2, Parameter3, resources, Parameter10, codeupdate, step_received, step_computed, dynamic_computed, step_sended, id_entity, id_project, id_type, name_type, color  mask(S-function:msfcn_unit_delay){Parameter1='Security_Cameras_Server_1', Parameter2=1, Parameter3='ORO', resources=, Parameter10=off, codeupdate=off, step_received=|, step_computed=, dynamic_computed=, step_sended=|, id_entity=159, id_project=6, id_type=40, name_type=App_Server, color=#00AAFF}
      mask step_received=|
      | Connection=max(Connection_init,TLC_CONN);
      | TLC_services=max(TLC_services_init,TLC_SERVICE);
      | TLC_services=mod(TLC_services,10);
      | TLC_revoke=floor(TLC_SERVICE/10);
      |
      | Mechanical_Fault=max([Mechanical_Fault Mechanical_Fault_init]);
      |
      | %if strcmp(name_entity,"BlockChainServer") && (cisia.major_time>=2)
      |  % Dos_attack=1;
      |  %TLC_revoke(9)=1;
      |  %TLC_services(9)=0;
      | %end
      |
      |
      | Cyber_Fault=max(CYBER_FAULT, transpose([Dos_attack   MITM_attack Virus_Attack Port_Scan_Attack  BGP_hijacking BotNet_Attack Data_Corruption SW_Change Config_Change Port_Saturation]));
      |
      | Service_Fault=max(abs(Consumed_Services.*TLC_services-Consumed_Services));
      | Redundancy_Fault=max(abs(Consumed_Services.*TLC_CONN-Consumed_Services));
      |
      | Conn_Fault=max([Dos_attack  Mechanical_Fault  1-POWER 1-ROOM_QoS] );
      |
      |
      | Operative_Level=(1-Conn_Fault)*(1-0.5*max(Cyber_Fault))*(1-Service_Fault)*max(max(TLC_CONN),0.5);
      mask step_sended=|
      | TLC_CONN=Connection*(1-Conn_Fault);
      | TLC_SERVICE=TLC_services*(1-Conn_Fault)*(1-Service_Fault)*(1-syslog_adm_login)+10*TLC_revoke;
      | CYBER_FAULT=Cyber_Fault*(1-Conn_Fault);
      mask prompts: Parameter1 "entity name"; Parameter2 "sampling time"; Parameter3 "project"; resources "input resources and state variables"; Parameter10 "Bring state variables to output"; codeupdate "update code from mask"
      mask help: This is a level-2 MATLAB file S-function which demonstrates CISIA entity
      mask DialogControl Container1 Prompt: All parameters
      mask Display: image('Icons/App_Server.png')
  Splitter_1 (54) : M-S-Function  FunctionName=cisia_msfun  Parameters=Parameter1, Parameter2, Parameter3, resources, Parameter10, codeupdate, step_received, step_computed, dynamic_computed, step_sended, id_entity, id_project, id_type, name_type, color  mask(S-function:msfcn_unit_delay){Parameter1='Splitter_1', Parameter2=1, Parameter3='ORO', resources=, Parameter10=off, codeupdate=off, step_received=|, step_computed=, dynamic_computed=, step_sended=|, id_entity=54, id_project=6, id_type=11, name_type=Splitter, color=#90DB5A}
      mask step_received=|
      | Connection=max(Connection_init,NGPON_CONN);
      | TLC_services=max(TLC_services_init,TLC_SERVICE);
      | TLC_services=mod(TLC_services,10);
      | TLC_revoke=floor(TLC_SERVICE/10);
      |
      | Cyber_Fault=max(CYBER_FAULT, transpose([Dos_attack   MITM_attack Virus_Attack Port_Scan_Attack  BGP_hijacking BotNet_Attack Data_Corruption SW_Change Config_Change Port_Saturation]));
      |
      | % Vale 1 in presenza di fault
      | Conn_Fault=max([Dos_attack  Mechanical_Fault] );
      |
      | Operative_Level=(1-Conn_Fault)*max(max(NGPON_CONN),0.5)*(1-0.5*max(Cyber_Fault)) ;
      mask step_sended=|
      | NGPON_IN=Connection;
      |
      | NGPON_CONN=Connection*(1-Conn_Fault);
      | TLC_SERVICE=TLC_services*(1-Conn_Fault)+10*TLC_revoke;
      |
      | Cyber_Transmitted=min(Cyber_Fault, transpose([0 0 1 0 1 1 0 0 0 1]));
      | CYBER_FAULT=Cyber_Transmitted*(1-Conn_Fault);
      |
      |
      | ROUTING_QoS=Operative_Level;
      mask prompts: Parameter1 "entity name"; Parameter2 "sampling time"; Parameter3 "project"; resources "input resources and state variables"; Parameter10 "Bring state variables to output"; codeupdate "update code from mask"
      mask help: This is a level-2 MATLAB file S-function which demonstrates CISIA entity
      mask DialogControl Container1 Prompt: All parameters
      mask Display: disp('Splitter')
  Streamer_6 (77) : M-S-Function  FunctionName=cisia_msfun  Parameters=Parameter1, Parameter2, Parameter3, resources, Parameter10, codeupdate, step_received, step_computed, dynamic_computed, step_sended, id_entity, id_project, id_type, name_type, color  mask(S-function:msfcn_unit_delay){Parameter1='Streamer_6', Parameter2=1, Parameter3='ORO', resources=, Parameter10=off, codeupdate=off, step_received=|, step_computed=, dynamic_computed=, step_sended=|, id_entity=77, id_project=6, id_type=17, name_type=Streamer, color=#16C75D}
      mask step_received=|
      | Connection=Connection_init*STREAM(1);
      | TLC_services=TLC_services_init*STREAM(1);
      | TLC_services=mod(TLC_services,10);
      | Mechanical_Fault=max([Mechanical_Fault Mechanical_Fault_init]);
      |
      | Cyber_Fault=max(zeros(10,1), transpose([Dos_attack   MITM_attack Virus_Attack Port_Scan_Attack  BGP_hijacking BotNet_Attack Data_Corruption SW_Change Config_Change Port_Saturation]));
      |
      |
      | Conn_Fault=max([Dos_attack  Mechanical_Fault] );
      |
      | Service_Fault=0;
      | Redundancy_Fault=0;
      |
      | Operative_Level=(1-Conn_Fault)*(1-0.5*max(Cyber_Fault))*(1-Service_Fault);
      mask step_sended=|
      | TLC_CONN=Connection*(1-Conn_Fault);
      | TLC_SERVICE=TLC_services*(1-Conn_Fault)*(1-Service_Fault);
      | %TLC_SERVICE=TLC_services
      |
      | Cyber_Transmitted=min(Cyber_Fault, transpose([0 0 1 0 1 1 0 0 0 1]));
      | CYBER_FAULT=Cyber_Transmitted*(1-Conn_Fault);
      mask prompts: Parameter1 "entity name"; Parameter2 "sampling time"; Parameter3 "project"; resources "input resources and state variables"; Parameter10 "Bring state variables to output"; codeupdate "update code from mask"
      mask help: This is a level-2 MATLAB file S-function which demonstrates CISIA entity
      mask DialogControl Container1 Prompt: All parameters
      mask Display: image('Icons/Streamer.png')
  TV_2 (155) : M-S-Function  FunctionName=cisia_msfun  Parameters=Parameter1, Parameter2, Parameter3, resources, Parameter10, codeupdate, step_received, step_computed, dynamic_computed, step_sended, id_entity, id_project, id_type, name_type, color  mask(S-function:msfcn_unit_delay){Parameter1='TV_2', Parameter2=1, Parameter3='ORO', resources=, Parameter10=off, codeupdate=off, step_received=|, step_computed=, dynamic_computed=, step_sended=|, id_entity=155, id_project=6, id_type=19, name_type=Television, color=#90DB5A}
      mask step_received=|
      | Connection=ADSL_CONN;
      | TLC_services=max(TLC_services_init,TLC_SERVICE);
      | TLC_services=mod(TLC_services,10);
      | TLC_revoke=floor(TLC_SERVICE/10);
      |
      | Cyber_Fault=max(zeros(10,1), transpose([Dos_attack   MITM_attack Virus_Attack Port_Scan_Attack  BGP_hijacking BotNet_Attack Data_Corruption SW_Change Config_Change Port_Saturation]));
      |
      | Port_Isolation=min(max(transpose([1 1 1 1 1 1 1 1 1 0]), CYBER_FAULT));
      |
      | % Vale 1 in presenza di fault
      | Conn_Fault=max([Dos_attack  Mechanical_Fault] );
      |
      | Service_Fault=max(abs(Consumed_Services.*TLC_services-Consumed_Services));
      | Redundancy_Fault=max(abs(Consumed_Services.*ADSL_CONN-Consumed_Services));
      |
      |
      | Alt_Serv_Fault=max(abs(Alternative_Services.*ADSL_CONN-Alternative_Services));
      |
      | Alt_Rout_Fault=max(abs(Consumed_Services.*ADSL_CONN-Consumed_Services));
      |
      | Port_Isolation=min(max(transpose([1 1 1 1 1 1 1 1 1 0]), CYBER_FAULT));
      |
      |
      | Operative_Level=(1-Conn_Fault)*max(max(ADSL_CONN),0.5)*(((1-Service_Fault)+(1-Redundancy_Fault)+(1-Port_Isolation))/3);
      |
      | Alt_Port_Isol=(1-Conn_Fault)*max(max(ADSL_CONN),0.5)*(((1-Service_Fault)+(1-Redundancy_Fault))/2);
      |
      |
      |
      | % Il servizio utilizzato
      | My_Service=max([(1-Service_Fault) (1-Redundancy_Fault)/2]);
      mask step_sended=|
      | TV_QoS=My_Service;
      |
      | ALT_SERVICES=1-Alt_Serv_Fault;
      | ALT_ROUTING=1-Alt_Rout_Fault;
      | ALT_PORT_ISOLATION=Alt_Port_Isol;
      mask prompts: Parameter1 "entity name"; Parameter2 "sampling time"; Parameter3 "project"; resources "input resources and state variables"; Parameter10 "Bring state variables to output"; codeupdate "update code from mask"
      mask help: This is a level-2 MATLAB file S-function which demonstrates CISIA entity
      mask DialogControl Container1 Prompt: All parameters
      mask Display: image('Icons/Television.png')
  Tap (119) : M-S-Function  FunctionName=cisia_msfun  Parameters=Parameter1, Parameter2, Parameter3, resources, Parameter10, codeupdate, step_received, step_computed, dynamic_computed, step_sended, id_entity, id_project, id_type, name_type, color  mask(S-function:msfcn_unit_delay){Parameter1='Tap', Parameter2=1, Parameter3='ORO', resources=, Parameter10=off, codeupdate=off, step_received=Operative_Level=1-Mechanical_Fault;, step_computed=, dynamic_computed=, step_sended=WATER=1-Mechanical_Fault;, id_entity=119, id_project=6, id_type=30, name_type=Tap, color=#FFFFFF}
      mask prompts: Parameter1 "entity name"; Parameter2 "sampling time"; Parameter3 "project"; resources "input resources and state variables"; Parameter10 "Bring state variables to output"; codeupdate "update code from mask"
      mask help: This is a level-2 MATLAB file S-function which demonstrates CISIA entity
      mask DialogControl Container1 Prompt: All parameters
      mask Display: disp('Tap')
  VHF_1 (212) : M-S-Function  FunctionName=cisia_msfun  Parameters=Parameter1, Parameter2, Parameter3, resources, Parameter10, codeupdate, step_received, step_computed, dynamic_computed, step_sended, id_entity, id_project, id_type, name_type, color  mask(S-function:msfcn_unit_delay){Parameter1='VHF_1', Parameter2=1, Parameter3='ORO', resources=, Parameter10=off, codeupdate=off, step_received=|, step_computed=, dynamic_computed=, step_sended=|, id_entity=212, id_project=6, id_type=46, name_type=VDES_ANTENNA, color=#FFFFFF}
      mask step_received=|
      | Connection=max(Connection_init,TLC_CONN);
      | TLC_services=max(TLC_services_init,TLC_SERVICE);
      | TLC_services=mod(TLC_services,10);
      | TLC_revoke=floor(TLC_SERVICE/10);
      |
      | Cyber_Fault=max(CYBER_FAULT, transpose([Dos_attack   MITM_attack Virus_Attack Port_Scan_Attack  BGP_hijacking BotNet_Attack Data_Corruption SW_Change Config_Change Port_Saturation]));
      |
      | % Vale 1 in presenza di fault
      | Conn_Fault=max([Dos_attack  Mechanical_Fault  1-POWER 1-VDES_CONN] );
      |
      | Service_Fault=max(abs(Consumed_Services.*TLC_services-Consumed_Services));
      | Redundancy_Fault=max(abs(Consumed_Services.*TLC_CONN-Consumed_Services));
      |
      |
      | Operative_Level=(1-Conn_Fault)*max(max(TLC_CONN),0.5)*((2*(1-Service_Fault)+(1-Redundancy_Fault))/3);
      |
      | % Il servizio utilizzato
      | My_Service=max([(1-Service_Fault) (1-Redundancy_Fault)/2]);
      mask step_sended=|
      | VDES_CONN=(1-Service_Fault);
      | TLC_CONN=Connection*(1-Conn_Fault);
      | TLC_SERVICE=TLC_services*(1-Conn_Fault)*(1-Service_Fault)+10*TLC_revoke;
      |
      | Cyber_Transmitted=min(Cyber_Fault, transpose([0 0 1 0 1 1 0 0 0 1]));
      | CYBER_FAULT=Cyber_Transmitted*(1-Conn_Fault);
      mask prompts: Parameter1 "entity name"; Parameter2 "sampling time"; Parameter3 "project"; resources "input resources and state variables"; Parameter10 "Bring state variables to output"; codeupdate "update code from mask"
      mask help: This is a level-2 MATLAB file S-function which demonstrates CISIA entity
      mask DialogControl Container1 Prompt: All parameters
      mask Display: image('Icons/VDES_ANTENNA.png')
  Wire_15 (44) : M-S-Function  FunctionName=cisia_msfun  Parameters=Parameter1, Parameter2, Parameter3, resources, Parameter10, codeupdate, step_received, step_computed, dynamic_computed, step_sended, id_entity, id_project, id_type, name_type, color  mask(S-function:msfcn_unit_delay){Parameter1='Wire_15', Parameter2=1, Parameter3='ORO', resources=, Parameter10=off, codeupdate=off, step_received=|, step_computed=, dynamic_computed=, step_sended=|, id_entity=44, id_project=6, id_type=1, name_type=Optical_Wire, color=#99CCFF}
      mask step_received=|
      | Connection=max(Connection_init,TLC_CONN);
      | TLC_services=max(TLC_services_init,TLC_SERVICE);
      | TLC_services=mod(TLC_services,10);
      | TLC_revoke=floor(TLC_SERVICE/10);
      |
      | Cyber_Fault=CYBER_FAULT;
      |
      | Mechanical_Fault=max([Mechanical_Fault MECH_FAULT Mechanical_Fault_init]);
      |
      | %TLC_services=TLC_services.*(1-TLC_revoke);
      |
      | Operative_Level=1-Mechanical_Fault;
      mask step_sended=|
      | TLC_CONN=Connection*Operative_Level;
      | TLC_SERVICE=TLC_services*Operative_Level+TLC_revoke*10;
      |
      |
      | CYBER_FAULT=Cyber_Fault*Operative_Level;
      | MECH_FAULT=Mechanical_Fault;
      mask prompts: Parameter1 "entity name"; Parameter2 "sampling time"; Parameter3 "project"; resources "input resources and state variables"; Parameter10 "Bring state variables to output"; codeupdate "update code from mask"
      mask help: This is a level-2 MATLAB file S-function which demonstrates CISIA entity
      mask DialogControl Container1 Prompt: All parameters
      mask Display: image('Icons/Optical_Wire.png')
  Wire_15a (49) : M-S-Function  FunctionName=cisia_msfun  Parameters=Parameter1, Parameter2, Parameter3, resources, Parameter10, codeupdate, step_received, step_computed, dynamic_computed, step_sended, id_entity, id_project, id_type, name_type, color  mask(S-function:msfcn_unit_delay){Parameter1='Wire_15a', Parameter2=1, Parameter3='ORO', resources=, Parameter10=off, codeupdate=off, step_received=|, step_computed=, dynamic_computed=, step_sended=|, id_entity=49, id_project=6, id_type=1, name_type=Optical_Wire, color=#99CCFF}
      mask step_received=|
      | Connection=max(Connection_init,TLC_CONN);
      | TLC_services=max(TLC_services_init,TLC_SERVICE);
      | TLC_services=mod(TLC_services,10);
      | TLC_revoke=floor(TLC_SERVICE/10);
      |
      | Cyber_Fault=CYBER_FAULT;
      |
      | Mechanical_Fault=max([Mechanical_Fault MECH_FAULT Mechanical_Fault_init]);
      |
      | %TLC_services=TLC_services.*(1-TLC_revoke);
      |
      | Operative_Level=1-Mechanical_Fault;
      mask step_sended=|
      | TLC_CONN=Connection*Operative_Level;
      | TLC_SERVICE=TLC_services*Operative_Level+TLC_revoke*10;
      |
      |
      | CYBER_FAULT=Cyber_Fault*Operative_Level;
      | MECH_FAULT=Mechanical_Fault;
      mask prompts: Parameter1 "entity name"; Parameter2 "sampling time"; Parameter3 "project"; resources "input resources and state variables"; Parameter10 "Bring state variables to output"; codeupdate "update code from mask"
      mask help: This is a level-2 MATLAB file S-function which demonstrates CISIA entity
      mask DialogControl Container1 Prompt: All parameters
      mask Display: image('Icons/Optical_Wire.png')
  Wire_S_2 (167) : M-S-Function  FunctionName=cisia_msfun  Parameters=Parameter1, Parameter2, Parameter3, resources, Parameter10, codeupdate, step_received, step_computed, dynamic_computed, step_sended, id_entity, id_project, id_type, name_type, color  mask(S-function:msfcn_unit_delay){Parameter1='Wire_S_2', Parameter2=1, Parameter3='ORO', resources=, Parameter10=off, codeupdate=off, step_received=|, step_computed=, dynamic_computed=, step_sended=|, id_entity=167, id_project=6, id_type=29, name_type=Wire_Medical_Room, color=#FFDD00}
      mask step_received=|
      | Power_Fault=1-POWER;
      |
      | Operative_Level = (1-Mechanical_Fault)*(1-0.5*Power_Fault);
      mask step_sended=|
      | POWER=Operative_Level;
      | WIRE_QoS=Operative_Level;
      mask prompts: Parameter1 "entity name"; Parameter2 "sampling time"; Parameter3 "project"; resources "input resources and state variables"; Parameter10 "Bring state variables to output"; codeupdate "update code from mask"
      mask help: This is a level-2 MATLAB file S-function which demonstrates CISIA entity
      mask DialogControl Container1 Prompt: All parameters
      mask Display: disp('Wire_Medical_Room')
  Woods_1 (305) : M-S-Function  FunctionName=cisia_msfun  Parameters=Parameter1, Parameter2, Parameter3, resources, Parameter10, codeupdate, step_received, step_computed, dynamic_computed, step_sended, id_entity, id_project, id_type, name_type, color  mask(S-function:msfcn_unit_delay){Parameter1='Woods_1', Parameter2=1, Parameter3='ORO', resources=, Parameter10=off, codeupdate=off, step_received=|, step_computed=, dynamic_computed=, step_sended=|, id_entity=305, id_project=6, id_type=65, name_type=Forest, color=#FFFFFF}
      mask step_received=|
      | Operative_Level=(1-Fire_Fault)*max(PLANE_QoS, 0.5);
      |
      | WOODS_HEALTH=Operative_Level;
      mask step_sended=|
      | FLAME=Fire_Fault;
      | WOODS_HEALTH=Operative_Level;
      mask prompts: Parameter1 "entity name"; Parameter2 "sampling time"; Parameter3 "project"; resources "input resources and state variables"; Parameter10 "Bring state variables to output"; codeupdate "update code from mask"
      mask help: This is a level-2 MATLAB file S-function which demonstrates CISIA entity
      mask DialogControl Container1 Prompt: All parameters
      mask Display: image('Icons/Forest.png')
  wires:
  Wire_15 (44)/4 -> Wire_15a (49)/4  "MECH_FAULT"
  Wire_15a (49)/4 -> Wire_15 (44)/4  "MECH_FAULT"
  CISIA_MASTER (0)/3 -> Display20/1  "DELTA TIME"
  CISIA_MASTER (0)/2 -> Display19/1  "MAJOR HITS"
  CISIA_MASTER (0)/4 -> Display21/1  "TIME PAST"
  CISIA_MASTER (0)/1 -> Display18/1  "MINOR HITS"
